simulink model "gm_uz_ninephase_VSD_transformation"  (R2021b)
settings: Solver=FixedStepAuto  StartTime=0.0  StopTime=inf  RelTol=1e-3
undefined symbols (not defined in the file or in its folder): a, b, c
libraries: hdlsllib x90, simulink x32, hdlmdlgenlib x20, dspsigops x7
(part 2 of 6)

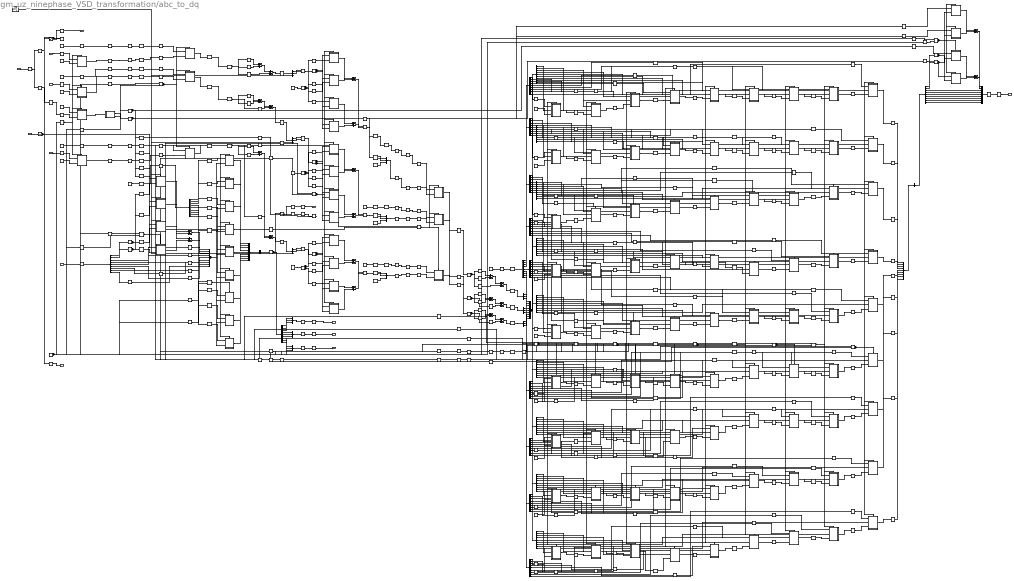
== system gm_uz_ninephase_VSD_transformation/abc_to_dq ==
  note: sin/cos calculation
  note: VSD and Park transformation
  note: VSD and Park inverse transformation
  note: Trigger Output
  x_in_dq : Inport  OutDataTypeStr=fixdt(1, 27, 18)  PortDimensions=[9]  SampleTime=1e-08
  theta_el : Inport  Port=2  OutDataTypeStr=fixdt(1, 18, 14)  PortDimensions=1  SampleTime=1e-08
  trigger_new_values : Inport  Port=3  OutDataTypeStr=boolean  PortDimensions=1  SampleTime=1e-08
  x_abc1_ll_pl : Inport  Port=4  OutDataTypeStr=fixdt(1, 27, 16)  PortDimensions=[3]  SampleTime=1e-08
  x_abc2_ll_pl : Inport  Port=5  OutDataTypeStr=fixdt(1, 27, 16)  PortDimensions=[3]  SampleTime=1e-08
  x_abc3_ll_pl : Inport  Port=6  OutDataTypeStr=fixdt(1, 27, 16)  PortDimensions=[3]  SampleTime=1e-08
  Add : Sum  AccumDataTypeStr=fixdt(1, 28, 16)  OutDataTypeStr=fixdt(1, 27, 16)  SampleTime=1e-10
  Add1 : Sum  AccumDataTypeStr=fixdt(1, 28, 18)  OutDataTypeStr=fixdt(1, 27, 18)  SampleTime=1e-10
  Add11 : Sum  Inputs=+-  AccumDataTypeStr=fixdt(1, 28, 16)  OutDataTypeStr=fixdt(1, 27, 16)  SampleTime=1e-10
  Add2 : Sum  Inputs=+-  AccumDataTypeStr=fixdt(1, 28, 18)  OutDataTypeStr=fixdt(1, 27, 18)  SampleTime=1e-10
  Complex to Real-Imag : ComplexToRealImag  SampleTime=1e-10
  Complex to Real-Imag1 : ComplexToRealImag  SampleTime=1e-10
  Complex to Real-Imag2 : ComplexToRealImag  SampleTime=1e-10
  Constant : Constant  Value=0  OutDataTypeStr=fixdt(1, 27, 16)  SampleTime=1e-10
  Constant1 : Constant  Value=[1;-0.5;-0.5;0.939697265625;-0.7660369873046875;-0.17364501953125;0.7660369873046875;-0.939697265625;0.17364501953125;0;0.86602783203125;-0.86602783203125;0.3420257568359375;0.642791748046875;-0.98480224609375;0.642791748046875;0.3420257568359375;-0.98480224609375;1;1;1;0.5;0.5;0.5;-0.5;-0.5;-0.5;0;0;0;0.86602783203125;0.86602783203125;0.86602783203125;0.86602783203125;0.86602783203125;0.86602783203125;1;-0.5;-0.5;-0.17364501953125;0.939697265625;-0.7660369873046875;-0.939697265625;0.17364501953125;0.7660369873046875;0;-0.86602783203125;0.86602783203125;0.98480224609375;-0.3420257568359375;-0.642791748046875;-0.3420257568359375;0.98480224609375;-0.642791748046875;1;-0.5;-0.5;-0.7660369873046875;-0.17364501953125;0.939697265625;0.17364501953125;0.7660369873046875;-0.939697265625;0;0.86602783203125;-0.86602783203125;0.642791748046875;-0.98480224609375;0.3420257568359375;-0.98480224609375;0.642791748046875;0.3420257568359375;1;1;1;-1;-1;-1;1;1;1]  OutDataTypeStr=fixdt(1, 18, 16)  SampleTime=1e-10
  Constant11 : Constant  Value=[0.22222137451171875;0;0.22222137451171875;0;0.22222137451171875;0;0.22222137451171875;0;0.111114501953125;-0.111114501953125;0.19245147705078125;0.22222137451171875;0;-0.111114501953125;-0.19245147705078125;-0.111114501953125;0.19245147705078125;0.111114501953125;-0.111114501953125;-0.19245147705078125;0.22222137451171875;0;-0.111114501953125;0.19245147705078125;-0.111114501953125;-0.19245147705078125;0.111114501953125;0.20882415771484375;0.0760040283203125;0.111114501953125;0.19245147705078125;-0.0385894775390625;0.21884918212890625;-0.17023468017578125;0.14284515380859375;-0.111114501953125;-0.17023468017578125;0.14284515380859375;0.111114501953125;0.19245147705078125;0.20882415771484375;-0.0760040283203125;-0.0385894775390625;-0.21884918212890625;-0.111114501953125;-0.0385894775390625;-0.21884918212890625;0.111114501953125;0.19245147705078125;-0.17023468017578125;-0.14284515380859375;0.20882415771484375;0.0760040283203125;-0.111114501953125;0.17023468017578125;0.14284515380859375;-0.111114501953125;0.19245147705078125;-0.20882415771484375;-0.0760040283203125;0.0385894775390625;-0.21884918212890625;0.111114501953125;-0.20882415771484375;0.0760040283203125;-0.111114501953125;0.19245147705078125;0.0385894775390625;0.21884918212890625;0.17023468017578125;0.14284515380859375;0.111114501953125;0.0385894775390625;-0.21884918212890625;-0.111114501953125;0.19245147705078125;0.17023468017578125;-0.14284515380859375;-0.20882415771484375;0.0760040283203125;0.111114501953125]  OutDataTypeStr=fixdt(1, 18, 17)  SampleTime=1e-10
  Constant12 : Constant  Value="fi(0,1,18,16,\"hex\",\"08000 + 3b619 i\")"  OutDataTypeStr=fixdt(1, 18, 16)  SampleTime=1e-10
  Constant13 : Constant  Value="fi(0,1,18,16,\"hex\",\"08000 + 3b619 i\")"  OutDataTypeStr=fixdt(1, 18, 16)  SampleTime=1e-10
  Constant14 : Constant  Value="fi(0,1,18,16,\"hex\",\"08000 + 3b619 i\")"  OutDataTypeStr=fixdt(1, 18, 16)  SampleTime=1e-10
  Constant2 : Constant  Value=0  OutDataTypeStr=fixdt(1, 27, 16)  SampleTime=1e-10
  Constant3 : Constant  Value=0  OutDataTypeStr=fixdt(1, 27, 16)  SampleTime=1e-10
  Delay9 : RateTransition  OutPortSampleTimeOpt=Multiple of input port sample time  OutPortSampleTimeMultiple=100
  Demux1_mux_1 : Mux  Inputs=3
  Demux1_mux_2 : Mux  Inputs=3
  Demux1_mux_3 : Mux  Inputs=3
  Demux1_out1 : Delay  DelayLength=double(1)  InitialCondition=0  SampleTime=1e-10
  Demux1_out2 : Delay  DelayLength=double(1)  InitialCondition=0  SampleTime=1e-10
  Demux1_out3 : Delay  DelayLength=double(1)  InitialCondition=0  SampleTime=1e-10
  Divide : Subsystem
      settings: MinAlgLoopOccurrences=on
  Divide1 : Subsystem
      settings: MinAlgLoopOccurrences=on
  Divide11 : Subsystem
      settings: MinAlgLoopOccurrences=on
  Divide2 : Subsystem
      settings: MinAlgLoopOccurrences=on
  Divide21 : Subsystem
      settings: MinAlgLoopOccurrences=on
  Divide3 : Subsystem
      settings: MinAlgLoopOccurrences=on
  Divide31 : Subsystem
      settings: MinAlgLoopOccurrences=on
  Divide4 : Subsystem
      settings: MinAlgLoopOccurrences=on
  From{,1..3,11..12,17..18,21..22} (10 alike) : hdlmdlgenlib/Buffer
      settings: SourceProductBaseCode=SL
  Gain : Subsystem
      settings: MinAlgLoopOccurrences=on
  Gain2 : Subsystem
      settings: MinAlgLoopOccurrences=on
  Gain21 : Subsystem
      settings: MinAlgLoopOccurrences=on
  Gain22 : Subsystem
      settings: MinAlgLoopOccurrences=on
  Gain2_const : Constant  Value=0.6666717529296875  OutDataTypeStr=fixdt(1, 18, 16)  SampleTime=1e-10
  Gain2_const1 : Constant  Value=0.6666717529296875  OutDataTypeStr=fixdt(1, 18, 16)  SampleTime=1e-10
  Gain2_const2 : Constant  Value=0.6666717529296875  OutDataTypeStr=fixdt(1, 18, 16)  SampleTime=1e-10
  Gain2_out_dtc : DataTypeConversion  OutDataTypeStr=fixdt(1, 27, 16)  SampleTime=1e-10  SaturateOnIntegerOverflow=on
  Gain2_out_dtc1 : DataTypeConversion  OutDataTypeStr=fixdt(1, 27, 16)  SampleTime=1e-10  SaturateOnIntegerOverflow=on
  Gain2_out_dtc2 : DataTypeConversion  OutDataTypeStr=fixdt(1, 27, 16)  SampleTime=1e-10  SaturateOnIntegerOverflow=on
  Gain4_const : Constant  Value=[1;0;0.5;-0.5;0.86602783203125;0.5;-0.5;-0.86602783203125;0.5]  OutDataTypeStr=fixdt(1, 18, 16)  SampleTime=1e-10
  Gain4_const1 : Constant  Value=[1;-0.5;-0.5;0;0.86602783203125;-0.86602783203125;1;1;1]  OutDataTypeStr=fixdt(1, 18, 16)  SampleTime=1e-10
  Gain4_const2 : Constant  Value=[1;0;0.5;-0.5;0.86602783203125;0.5;-0.5;-0.86602783203125;0.5]  OutDataTypeStr=fixdt(1, 18, 16)  SampleTime=1e-10
  Gain4_const3 : Constant  Value=[1;-0.5;-0.5;0;0.86602783203125;-0.86602783203125;1;1;1]  OutDataTypeStr=fixdt(1, 18, 16)  SampleTime=1e-10
  Gain4_const4 : Constant  Value=[1;0;0.5;-0.5;0.86602783203125;0.5;-0.5;-0.86602783203125;0.5]  OutDataTypeStr=fixdt(1, 18, 16)  SampleTime=1e-10
  Gain4_const5 : Constant  Value=[1;-0.5;-0.5;0;0.86602783203125;-0.86602783203125;1;1;1]  OutDataTypeStr=fixdt(1, 18, 16)  SampleTime=1e-10
  Gain_const : Constant  Value=0.1591548919677734375  OutDataTypeStr=fixdt(1, 18, 19)  SampleTime=1e-10
  Goto : hdlmdlgenlib/Buffer
      settings: SourceProductBaseCode=SL
  Goto1 : hdlmdlgenlib/Buffer
      settings: SourceProductBaseCode=SL
  Goto2 : hdlmdlgenlib/Buffer
      settings: SourceProductBaseCode=SL
  MMul_add_01 : Sum  OutDataTypeStr=fixdt(1, 27, 16)  SaturateOnIntegerOverflow=on  SampleTime=1e-10
  MMul_add_011 : Sum  OutDataTypeStr=fixdt(1, 27, 16)  SaturateOnIntegerOverflow=on  SampleTime=1e-10
  MMul_add_012 : Sum  OutDataTypeStr=fixdt(1, 27, 16)  SaturateOnIntegerOverflow=on  SampleTime=1e-10
  MMul_add_013 : Sum  OutDataTypeStr=fixdt(1, 27, 16)  SaturateOnIntegerOverflow=on  SampleTime=1e-10
  MMul_add_014 : Sum  OutDataTypeStr=fixdt(1, 27, 16)  SaturateOnIntegerOverflow=on  SampleTime=1e-10
  MMul_add_015 : Sum  OutDataTypeStr=fixdt(1, 27, 16)  SaturateOnIntegerOverflow=on  SampleTime=1e-10
  MMul_add_{12,121..125} (6 alike) : Sum  OutDataTypeStr=fixdt(1, 27, 16)  SaturateOnIntegerOverflow=on  SampleTime=1e-10
  MMul_dot_product : Subsystem
      settings: MinAlgLoopOccurrences=on
  MMul_dot_product1 : Subsystem
      settings: MinAlgLoopOccurrences=on
  MMul_dot_product2 : Subsystem
      settings: MinAlgLoopOccurrences=on
  MMul_dot_product3 : Subsystem
      settings: MinAlgLoopOccurrences=on
  MMul_dot_product4 : Subsystem
      settings: MinAlgLoopOccurrences=on
  MMul_dot_product5 : Subsystem
      settings: MinAlgLoopOccurrences=on
  MMul_dot_product_out_dtc{,1..5} (6 alike) : DataTypeConversion  OutDataTypeStr=fixdt(1, 27, 16)  SampleTime=1e-10  SaturateOnIntegerOverflow=on
  MatrixMultiply_out1_0_wire : hdlmdlgenlib/Buffer
      settings: SourceProductBaseCode=SL
  MatrixMultiply_out1_1_wire : hdlmdlgenlib/Buffer
      settings: SourceProductBaseCode=SL
  Product : Subsystem
      settings: MinAlgLoopOccurrences=on
  Product1 : Subsystem
      settings: MinAlgLoopOccurrences=on
  Product10 : Subsystem
      settings: MinAlgLoopOccurrences=on
  Product11 : Subsystem
      settings: MinAlgLoopOccurrences=on
  Product2 : Subsystem
      settings: MinAlgLoopOccurrences=on
  Product3 : Subsystem
      settings: MinAlgLoopOccurrences=on
  Product4 : Subsystem
      settings: MinAlgLoopOccurrences=on
  Product5 : Subsystem
      settings: MinAlgLoopOccurrences=on
  Product6 : Subsystem
      settings: MinAlgLoopOccurrences=on
  Product7 : Subsystem
      settings: MinAlgLoopOccurrences=on
  Product8 : Subsystem
      settings: MinAlgLoopOccurrences=on
  Product9 : Subsystem
      settings: MinAlgLoopOccurrences=on
  Product_AC_minus_BD : Sum  Inputs=+-  OutDataTypeStr=fixdt(1, 27, 16)  SampleTime=1e-10
  Product_AC_minus_BD1 : Sum  Inputs=+-  OutDataTypeStr=fixdt(1, 27, 16)  SampleTime=1e-10
  Product_AC_minus_BD2 : Sum  Inputs=+-  OutDataTypeStr=fixdt(1, 27, 16)  SampleTime=1e-10
  Product_AD_plus_BC : Sum  OutDataTypeStr=fixdt(1, 27, 16)  SampleTime=1e-10
  Product_AD_plus_BC1 : Sum  OutDataTypeStr=fixdt(1, 27, 16)  SampleTime=1e-10
  Product_AD_plus_BC2 : Sum  OutDataTypeStr=fixdt(1, 27, 16)  SampleTime=1e-10
  Product_C2ReIm_{1..2,11..12,21..22} (6 alike) : ComplexToRealImag  SampleTime=1e-10
  Product_ReIm2Complex : RealImagToComplex  SampleTime=1e-10
  Product_ReIm2Complex1 : RealImagToComplex  SampleTime=1e-10
  Product_ReIm2Complex2 : RealImagToComplex  SampleTime=1e-10
  Real-Imag to Complex : RealImagToComplex  ConstantPart="fi(0,1,27,16,\"hex\",\"0000000\")"  SampleTime=1e-10
  Real-Imag to Complex1 : RealImagToComplex  ConstantPart="fi(0,1,27,16,\"hex\",\"0000000\")"  SampleTime=1e-10
  Real-Imag to Complex2 : RealImagToComplex  ConstantPart="fi(0,1,27,16,\"hex\",\"0000000\")"  SampleTime=1e-10
  Reshape{,1..5} (6 alike) : Reshape  OutputDimensionality=Column vector (2-D)
  Row2Col_in{0..1,11..15} (7 alike) : Reshape  OutputDimensionality=Column vector (2-D)
  Row2Col_in01 : Reshape  OutputDimensionality=Column vector (2-D)
  Row2Col_in02 : Reshape  OutputDimensionality=Column vector (2-D)
  Row2Col_in03 : Reshape  OutputDimensionality=Column vector (2-D)
  Row2Col_in04 : Reshape  OutputDimensionality=Column vector (2-D)
  Row2Col_in05 : Reshape  OutputDimensionality=Column vector (2-D)
  Sine HDL Optimized : Subsystem  mask(Sine and Cosine HDL optimized block){OutputFormula=sin(2*pi*u) and cos(2*pi*u), NumDataPoints=double(256), TableDataTypeStr=fixdt(0,17,16), SimulateLUTROMDelay=off}
      mask prompts: OutputFormula "Simulink:masks:OutputFormula_MP"; NumDataPoints "HDLShared:hdlshared:CosineHDL_Npts"; TableDataTypeStr "Simulink:blkprm_prompts:TABLE_UNIFIEDDATATYPE"; SimulateLUTROMDelay "HDLShared:hdlshared:CosineHDL_SimulateLUTDelay"
      mask help: Sine and Cosine HDL optimized block using quarter wave symmetry, and HDL friendly settings.
      mask Help: helpview([docroot '/hdlcoder/helptargets.map'],'SineAndCosineHDL_Optimized');
      mask TypeOptions OutputFormula: sin(2*pi*u) | cos(2*pi*u) | exp(j*2*pi*u) | sin(2*pi*u) and cos(2*pi*u)
      mask Display:
      | port_label('input',1,'u')
      | port_label('output',1,'sin(2*pi*u)')
      | port_label('output',2,'cos(2*pi*u)')
      | xpos = 0.35;
      | yoffset = 0.5;
      | if ( SimulateLUTROMDelay )
      |   text(xpos,yoffset,'HDL (Z^{-1})','texmode','on')
      | else
      |    text(xpos,yoffset,'HDL')
      | end
  Switch : Switch  Criteria=u2 ~= 0  Threshold=double(0)  OutDataTypeStr=fixdt(1, 27, 18)  SampleTime=1e-10
  Switch1 : Switch  Criteria=u2 ~= 0  Threshold=double(0)  OutDataTypeStr=fixdt(1, 18, 14)  SampleTime=1e-08
  Switch_out1 : Delay  DelayLength=double(1)  InitialCondition=0  SampleTime=1e-10
  Switch_out11 : Delay  DelayLength=double(1)  InitialCondition=0  SampleTime=1e-10
  Transformation_out1 : Delay  DelayLength=double(1)  InitialCondition=0  SampleTime=1e-10
  Unit Delay : UnitDelay  SampleTime=1e-08
  _adder_MultiplyAdd : Subsystem
      settings: MinAlgLoopOccurrences=on
  _adder_MultiplyAdd1 : Subsystem
      settings: MinAlgLoopOccurrences=on
  _adder_MultiplyAdd10 : Subsystem
      settings: MinAlgLoopOccurrences=on
  _adder_MultiplyAdd11 : Subsystem
      settings: MinAlgLoopOccurrences=on
  _adder_MultiplyAdd12 : Subsystem
      settings: MinAlgLoopOccurrences=on
  _adder_MultiplyAdd13 : Subsystem
      settings: MinAlgLoopOccurrences=on
  _adder_MultiplyAdd14 : Subsystem
      settings: MinAlgLoopOccurrences=on
  _adder_MultiplyAdd15 : Subsystem
      settings: MinAlgLoopOccurrences=on
  _adder_MultiplyAdd16 : Subsystem
      settings: MinAlgLoopOccurrences=on
  _adder_MultiplyAdd17 : Subsystem
      settings: MinAlgLoopOccurrences=on
  _adder_MultiplyAdd18 : Subsystem
      settings: MinAlgLoopOccurrences=on
  _adder_MultiplyAdd19 : Subsystem
      settings: MinAlgLoopOccurrences=on
  _adder_MultiplyAdd2 : Subsystem
      settings: MinAlgLoopOccurrences=on
  _adder_MultiplyAdd20 : Subsystem
      settings: MinAlgLoopOccurrences=on
  _adder_MultiplyAdd21 : Subsystem
      settings: MinAlgLoopOccurrences=on
  _adder_MultiplyAdd22 : Subsystem
      settings: MinAlgLoopOccurrences=on
  _adder_MultiplyAdd23 : Subsystem
      settings: MinAlgLoopOccurrences=on
  _adder_MultiplyAdd24 : Subsystem
      settings: MinAlgLoopOccurrences=on
  _adder_MultiplyAdd25 : Subsystem
      settings: MinAlgLoopOccurrences=on
  _adder_MultiplyAdd26 : Subsystem
      settings: MinAlgLoopOccurrences=on
  _adder_MultiplyAdd27 : Subsystem
      settings: MinAlgLoopOccurrences=on
  _adder_MultiplyAdd28 : Subsystem
      settings: MinAlgLoopOccurrences=on
  _adder_MultiplyAdd29 : Subsystem
      settings: MinAlgLoopOccurrences=on
  _adder_MultiplyAdd3 : Subsystem
      settings: MinAlgLoopOccurrences=on
  _adder_MultiplyAdd30 : Subsystem
      settings: MinAlgLoopOccurrences=on
  _adder_MultiplyAdd31 : Subsystem
      settings: MinAlgLoopOccurrences=on
  _adder_MultiplyAdd32 : Subsystem
      settings: MinAlgLoopOccurrences=on
  _adder_MultiplyAdd33 : Subsystem
      settings: MinAlgLoopOccurrences=on
  _adder_MultiplyAdd34 : Subsystem
      settings: MinAlgLoopOccurrences=on
  _adder_MultiplyAdd35 : Subsystem
      settings: MinAlgLoopOccurrences=on
  _adder_MultiplyAdd36 : Subsystem
      settings: MinAlgLoopOccurrences=on
  _adder_MultiplyAdd37 : Subsystem
      settings: MinAlgLoopOccurrences=on
  _adder_MultiplyAdd38 : Subsystem
      settings: MinAlgLoopOccurrences=on
  _adder_MultiplyAdd39 : Subsystem
      settings: MinAlgLoopOccurrences=on
  _adder_MultiplyAdd4 : Subsystem
      settings: MinAlgLoopOccurrences=on
  _adder_MultiplyAdd40 : Subsystem
      settings: MinAlgLoopOccurrences=on
  _adder_MultiplyAdd41 : Subsystem
      settings: MinAlgLoopOccurrences=on
  _adder_MultiplyAdd42 : Subsystem
      settings: MinAlgLoopOccurrences=on
  _adder_MultiplyAdd43 : Subsystem
      settings: MinAlgLoopOccurrences=on
  _adder_MultiplyAdd44 : Subsystem
      settings: MinAlgLoopOccurrences=on
  _adder_MultiplyAdd45 : Subsystem
      settings: MinAlgLoopOccurrences=on
  _adder_MultiplyAdd46 : Subsystem
      settings: MinAlgLoopOccurrences=on
  _adder_MultiplyAdd47 : Subsystem
      settings: MinAlgLoopOccurrences=on
  _adder_MultiplyAdd48 : Subsystem
      settings: MinAlgLoopOccurrences=on
  _adder_MultiplyAdd49 : Subsystem
      settings: MinAlgLoopOccurrences=on
  _adder_MultiplyAdd5 : Subsystem
      settings: MinAlgLoopOccurrences=on
  _adder_MultiplyAdd50 : Subsystem
      settings: MinAlgLoopOccurrences=on
  _adder_MultiplyAdd51 : Subsystem
      settings: MinAlgLoopOccurrences=on
  _adder_MultiplyAdd52 : Subsystem
      settings: MinAlgLoopOccurrences=on
  _adder_MultiplyAdd53 : Subsystem
      settings: MinAlgLoopOccurrences=on
  _adder_MultiplyAdd54 : Subsystem
      settings: MinAlgLoopOccurrences=on
  _adder_MultiplyAdd55 : Subsystem
      settings: MinAlgLoopOccurrences=on
  _adder_MultiplyAdd56 : Subsystem
      settings: MinAlgLoopOccurrences=on
  _adder_MultiplyAdd57 : Subsystem
      settings: MinAlgLoopOccurrences=on
  _adder_MultiplyAdd58 : Subsystem
      settings: MinAlgLoopOccurrences=on
  _adder_MultiplyAdd59 : Subsystem
      settings: MinAlgLoopOccurrences=on
  _adder_MultiplyAdd6 : Subsystem
      settings: MinAlgLoopOccurrences=on
  _adder_MultiplyAdd60 : Subsystem
      settings: MinAlgLoopOccurrences=on
  _adder_MultiplyAdd61 : Subsystem
      settings: MinAlgLoopOccurrences=on
  _adder_MultiplyAdd62 : Subsystem
      settings: MinAlgLoopOccurrences=on
  _adder_MultiplyAdd63 : Subsystem
      settings: MinAlgLoopOccurrences=on
  _adder_MultiplyAdd64 : Subsystem
      settings: MinAlgLoopOccurrences=on
  _adder_MultiplyAdd65 : Subsystem
      settings: MinAlgLoopOccurrences=on
  _adder_MultiplyAdd66 : Subsystem
      settings: MinAlgLoopOccurrences=on
  _adder_MultiplyAdd67 : Subsystem
      settings: MinAlgLoopOccurrences=on
  _adder_MultiplyAdd68 : Subsystem
      settings: MinAlgLoopOccurrences=on
  _adder_MultiplyAdd69 : Subsystem
      settings: MinAlgLoopOccurrences=on
  _adder_MultiplyAdd7 : Subsystem
      settings: MinAlgLoopOccurrences=on
  _adder_MultiplyAdd70 : Subsystem
      settings: MinAlgLoopOccurrences=on
  _adder_MultiplyAdd71 : Subsystem
      settings: MinAlgLoopOccurrences=on
  _adder_MultiplyAdd72 : Subsystem
      settings: MinAlgLoopOccurrences=on
  _adder_MultiplyAdd73 : Subsystem
      settings: MinAlgLoopOccurrences=on
  _adder_MultiplyAdd74 : Subsystem
      settings: MinAlgLoopOccurrences=on
  _adder_MultiplyAdd75 : Subsystem
      settings: MinAlgLoopOccurrences=on
  _adder_MultiplyAdd76 : Subsystem
      settings: MinAlgLoopOccurrences=on
  _adder_MultiplyAdd77 : Subsystem
      settings: MinAlgLoopOccurrences=on
  _adder_MultiplyAdd78 : Subsystem
      settings: MinAlgLoopOccurrences=on
  _adder_MultiplyAdd79 : Subsystem
      settings: MinAlgLoopOccurrences=on
  _adder_MultiplyAdd8 : Subsystem
      settings: MinAlgLoopOccurrences=on
  _adder_MultiplyAdd80 : Subsystem
      settings: MinAlgLoopOccurrences=on
  _adder_MultiplyAdd9 : Subsystem
      settings: MinAlgLoopOccurrences=on
  _adder_MultiplyAdd_out_dtc{,1..80} (81 alike) : DataTypeConversion  OutDataTypeStr=fixdt(1, 27, 16)  SampleTime=1e-10
  _bias{,1..8} (9 alike) : Constant  Value=double(0)  OutDataTypeStr=fixdt(1, 27, 16)  SampleTime=1e-10
  abc   to   alpha_beta_0_out1_2_term2 : Terminator
  abc   to   alpha_beta_0_out1_2_term21 : Terminator
  abc   to   alpha_beta_0_out1_2_term22 : Terminator
  crp_temp_MAC : Subsystem
      settings: MinAlgLoopOccurrences=on
  crp_temp_MAC1 : Subsystem
      settings: MinAlgLoopOccurrences=on
  crp_temp_MAC2 : Subsystem
      settings: MinAlgLoopOccurrences=on
  crp_temp_MAC3 : Subsystem
      settings: MinAlgLoopOccurrences=on
  crp_temp_MAC4 : Subsystem
      settings: MinAlgLoopOccurrences=on
  crp_temp_MAC5 : Subsystem
      settings: MinAlgLoopOccurrences=on
  crp_temp_MAC6 : Subsystem
      settings: MinAlgLoopOccurrences=on
  crp_temp_MAC7 : Subsystem
      settings: MinAlgLoopOccurrences=on
  crp_temp_MAC8 : Subsystem
      settings: MinAlgLoopOccurrences=on
  ctr_99 : simulink/Sources/Counter Limited  uplimit=double(99)  tsamp=1e-10
  delayMatch{,1,121..122} (4 alike) : Delay  DelayLength=double(1)  InitialCondition=0  SampleTime=1e-08
  delayMatch{2..21,23..27,29..33,35..120} (116 alike) : Delay  DelayLength=double(1)  InitialCondition=0  SampleTime=1e-10
  delayMatch22 : Delay  DelayLength=double(2)  InitialCondition=0  SampleTime=1e-10
  delayMatch28 : Delay  DelayLength=double(2)  InitialCondition=0  SampleTime=1e-10
  delayMatch34 : Delay  DelayLength=double(2)  InitialCondition=0  SampleTime=1e-10
  enb_counter_ge_11 : simulink/Logic and Bit Operations/Compare To Constant  relop=>=  const=double(11)  OutDataTypeStr=boolean
  enb_counter_ge_11_and_enb_counter_le_14 : Logic  AllPortsSameDT=off  OutDataTypeStr=boolean  SampleTime=1e-10
  enb_counter_ge_14 : simulink/Logic and Bit Operations/Compare To Constant  relop=>=  const=double(14)  OutDataTypeStr=boolean
  enb_counter_ge_14_and_enb_counter_le_17 : Logic  AllPortsSameDT=off  OutDataTypeStr=boolean  SampleTime=1e-10
  enb_counter_ge_17 : simulink/Logic and Bit Operations/Compare To Constant  relop=>=  const=double(17)  OutDataTypeStr=boolean
  enb_counter_ge_17_and_enb_counter_le_20 : Logic  AllPortsSameDT=off  OutDataTypeStr=boolean  SampleTime=1e-10
  enb_counter_ge_2 : simulink/Logic and Bit Operations/Compare To Constant  relop=>=  const=double(2)  OutDataTypeStr=boolean
  enb_counter_ge_20 : simulink/Logic and Bit Operations/Compare To Constant  relop=>=  const=double(20)  OutDataTypeStr=boolean
  enb_counter_ge_20_and_enb_counter_le_23 : Logic  AllPortsSameDT=off  OutDataTypeStr=boolean  SampleTime=1e-10
  enb_counter_ge_23 : simulink/Logic and Bit Operations/Compare To Constant  relop=>=  const=double(23)  OutDataTypeStr=boolean
  enb_counter_ge_23_and_enb_counter_le_26 : Logic  AllPortsSameDT=off  OutDataTypeStr=boolean  SampleTime=1e-10
  enb_counter_ge_26 : simulink/Logic and Bit Operations/Compare To Constant  relop=>=  const=double(26)  OutDataTypeStr=boolean
  enb_counter_ge_26_and_enb_counter_le_29 : Logic  AllPortsSameDT=off  OutDataTypeStr=boolean  SampleTime=1e-10
  enb_counter_ge_29 : simulink/Logic and Bit Operations/Compare To Constant  relop=>=  const=double(29)  OutDataTypeStr=boolean
  enb_counter_ge_29_and_enb_counter_le_32 : Logic  AllPortsSameDT=off  OutDataTypeStr=boolean  SampleTime=1e-10
  enb_counter_ge_2_and_enb_counter_le_4 : Logic  AllPortsSameDT=off  OutDataTypeStr=boolean  SampleTime=1e-10
  enb_counter_ge_3 : simulink/Logic and Bit Operations/Compare To Constant  relop=>=  const=double(3)  OutDataTypeStr=boolean
  enb_counter_ge_32 : simulink/Logic and Bit Operations/Compare To Constant  relop=>=  const=double(32)  OutDataTypeStr=boolean
  enb_counter_ge_32_and_enb_counter_le_35 : Logic  AllPortsSameDT=off  OutDataTypeStr=boolean  SampleTime=1e-10
  enb_counter_ge_35 : simulink/Logic and Bit Operations/Compare To Constant  relop=>=  const=double(35)  OutDataTypeStr=boolean
  enb_counter_ge_35_and_enb_counter_le_37 : Logic  AllPortsSameDT=off  OutDataTypeStr=boolean  SampleTime=1e-10
  enb_counter_ge_3_and_enb_counter_le_5 : Logic  AllPortsSameDT=off  OutDataTypeStr=boolean  SampleTime=1e-10
  enb_counter_ge_4 : simulink/Logic and Bit Operations/Compare To Constant  relop=>=  const=double(4)  OutDataTypeStr=boolean
  enb_counter_ge_4_and_enb_counter_le_6 : Logic  AllPortsSameDT=off  OutDataTypeStr=boolean  SampleTime=1e-10
  enb_counter_ge_5 : simulink/Logic and Bit Operations/Compare To Constant  relop=>=  const=double(5)  OutDataTypeStr=boolean
  enb_counter_ge_5_and_enb_counter_le_13 : Logic  AllPortsSameDT=off  OutDataTypeStr=boolean  SampleTime=1e-10
  enb_counter_ge_6 : simulink/Logic and Bit Operations/Compare To Constant  relop=>=  const=double(6)  OutDataTypeStr=boolean
  enb_counter_ge_6_and_enb_counter_le_8 : Logic  AllPortsSameDT=off  OutDataTypeStr=boolean  SampleTime=1e-10
  enb_counter_ge_8 : simulink/Logic and Bit Operations/Compare To Constant  relop=>=  const=double(8)  OutDataTypeStr=boolean
  enb_counter_ge_8_and_enb_counter_le_11 : Logic  AllPortsSameDT=off  OutDataTypeStr=boolean  SampleTime=1e-10
  enb_counter_le_11 : simulink/Logic and Bit Operations/Compare To Constant  relop=<=  const=double(11)  OutDataTypeStr=boolean
  enb_counter_le_13 : simulink/Logic and Bit Operations/Compare To Constant  relop=<=  const=double(13)  OutDataTypeStr=boolean
  enb_counter_le_14 : simulink/Logic and Bit Operations/Compare To Constant  relop=<=  const=double(14)  OutDataTypeStr=boolean
  enb_counter_le_17 : simulink/Logic and Bit Operations/Compare To Constant  relop=<=  const=double(17)  OutDataTypeStr=boolean
  enb_counter_le_2 : simulink/Logic and Bit Operations/Compare To Constant  relop=<=  const=double(2)  OutDataTypeStr=boolean
  enb_counter_le_20 : simulink/Logic and Bit Operations/Compare To Constant  relop=<=  const=double(20)  OutDataTypeStr=boolean
  enb_counter_le_23 : simulink/Logic and Bit Operations/Compare To Constant  relop=<=  const=double(23)  OutDataTypeStr=boolean
  enb_counter_le_26 : simulink/Logic and Bit Operations/Compare To Constant  relop=<=  const=double(26)  OutDataTypeStr=boolean
  enb_counter_le_29 : simulink/Logic and Bit Operations/Compare To Constant  relop=<=  const=double(29)  OutDataTypeStr=boolean
  enb_counter_le_32 : simulink/Logic and Bit Operations/Compare To Constant  relop=<=  const=double(32)  OutDataTypeStr=boolean
  enb_counter_le_35 : simulink/Logic and Bit Operations/Compare To Constant  relop=<=  const=double(35)  OutDataTypeStr=boolean
  enb_counter_le_37 : simulink/Logic and Bit Operations/Compare To Constant  relop=<=  const=double(37)  OutDataTypeStr=boolean
  enb_counter_le_4 : simulink/Logic and Bit Operations/Compare To Constant  relop=<=  const=double(4)  OutDataTypeStr=boolean
  enb_counter_le_5 : simulink/Logic and Bit Operations/Compare To Constant  relop=<=  const=double(5)  OutDataTypeStr=boolean
  enb_counter_le_6 : simulink/Logic and Bit Operations/Compare To Constant  relop=<=  const=double(6)  OutDataTypeStr=boolean
  enb_counter_le_8 : simulink/Logic and Bit Operations/Compare To Constant  relop=<=  const=double(8)  OutDataTypeStr=boolean
  in0_repeat : dspsigops/Repeat  N=double(100)  RateOptions=Allow multirate processing  ic=0  mode=Unused parameter value
  in1_repeat : dspsigops/Repeat  N=double(100)  RateOptions=Allow multirate processing  ic=0  mode=Unused parameter value
  in2_repeat : dspsigops/Repeat  N=double(100)  RateOptions=Allow multirate processing  ic=0  mode=Unused parameter value
  in3_repeat : dspsigops/Repeat  N=double(100)  RateOptions=Allow multirate processing  ic=0  mode=Unused parameter value
  in4_repeat : dspsigops/Repeat  N=double(100)  RateOptions=Allow multirate processing  ic=0  mode=Unused parameter value
  in5_repeat : dspsigops/Repeat  N=double(100)  RateOptions=Allow multirate processing  ic=0  mode=Unused parameter value
  in6_repeat : dspsigops/Repeat  N=double(100)  RateOptions=Allow multirate processing  ic=0  mode=Unused parameter value
  inverse Transformation_out1 : hdlmdlgenlib/Buffer
      settings: SourceProductBaseCode=SL
  mux : Mux  Inputs=3
  mux1 : Mux  Inputs=3
  mux2 : Mux  Inputs=3
  mux3 : Mux  Inputs=9
  mux4 : Mux  Inputs=9
  mux5 : Mux  Inputs=9
  reshape_dotProduct{,1..5} (6 alike) : Reshape  OutputDimensionality=Customize  OutputDimensions=[3,3]
  reshape_mmulResult{,1..5} (6 alike) : Reshape  OutputDimensionality=Customize  OutputDimensions=[3,1]
  select_0 : Selector  NumberOfDimensions=2  SampleTime=1e-10  IndexOptions=Index vector (dialog),Select all  Indices=double(1),[]  OutputSizes=1
  select_01 : Selector  NumberOfDimensions=2  SampleTime=1e-10  IndexOptions=Index vector (dialog),Select all  Indices=double(1),[]  OutputSizes=1
  select_02 : Selector  NumberOfDimensions=2  SampleTime=1e-10  IndexOptions=Index vector (dialog),Select all  Indices=double(1),[]  OutputSizes=1
  select_03 : Selector  NumberOfDimensions=2  SampleTime=1e-10  IndexOptions=Index vector (dialog),Select all  Indices=double(1),[]  OutputSizes=1
  select_04 : Selector  NumberOfDimensions=2  SampleTime=1e-10  IndexOptions=Index vector (dialog),Select all  Indices=double(1),[]  OutputSizes=1
  select_05 : Selector  NumberOfDimensions=2  SampleTime=1e-10  IndexOptions=Index vector (dialog),Select all  Indices=double(1),[]  OutputSizes=1
  select_{1,11..15} (6 alike) : Selector  NumberOfDimensions=2  SampleTime=1e-10  IndexOptions=Index vector (dialog),Select all  Indices=double(2),[]  OutputSizes=1
  select_{2,21..25} (6 alike) : Selector  NumberOfDimensions=2  SampleTime=1e-10  IndexOptions=Index vector (dialog),Select all  Indices=double(3),[]  OutputSizes=1
  select_indices0 : Selector  SampleTime=1e-10  IndexOptions=Index vector (dialog)  Indices=double([1 4 7 2 5 8 3 6 9])  OutputSizes=1
  select_indices01 : Selector  SampleTime=1e-10  IndexOptions=Index vector (dialog)  Indices=double([1 4 7 2 5 8 3 6 9])  OutputSizes=1
  select_indices02 : Selector  SampleTime=1e-10  IndexOptions=Index vector (dialog)  Indices=double([1 4 7 2 5 8 3 6 9])  OutputSizes=1
  select_indices03 : Selector  SampleTime=1e-10  IndexOptions=Index vector (dialog)  Indices=double([1 4 7 2 5 8 3 6 9])  OutputSizes=1
  select_indices04 : Selector  SampleTime=1e-10  IndexOptions=Index vector (dialog)  Indices=double([1 4 7 2 5 8 3 6 9])  OutputSizes=1
  select_indices05 : Selector  SampleTime=1e-10  IndexOptions=Index vector (dialog)  Indices=double([1 4 7 2 5 8 3 6 9])  OutputSizes=1
  select_indices{1,11..15} (6 alike) : Selector  SampleTime=1e-10  IndexOptions=Index vector (dialog)  Indices=double([1 2 3 1 2 3 1 2 3])  OutputSizes=1
  t{,7..8,25..42} (21 alike) : Demux  Outputs=9
  t{1..6} (6 alike) : Demux  Outputs=3
  t10 : Reshape  OutputDimensionality=Customize  OutputDimensions=[9,9]
  t{11..16} (6 alike) : Reshape  OutputDimensionality=Customize  OutputDimensions=[3,3]
  t17 : Math  Operator=transpose  SaturateOnIntegerOverflow=on
  t18 : Subsystem
  t19 : Mux  Inputs=9
  t20 : Concatenate  NumInputs=1  Mode=Multidimensional array  ConcatenateDimension=2
  t21 : Math  Operator=transpose  SaturateOnIntegerOverflow=on
  t22 : Subsystem
  t23 : Mux  Inputs=9
  t24 : Concatenate  NumInputs=1  Mode=Multidimensional array  ConcatenateDimension=2
  t{43..47} (5 alike) : RateTransition  OutPortSampleTimeOpt=Multiple of input port sample time  OutPortSampleTimeMultiple=100
  t9 : Reshape  OutputDimensionality=Customize  OutputDimensions=[9,9]
  vectorized_in0 : Reshape  OutputDimensionality=Row vector (2-D)
  vectorized_in01 : Reshape  OutputDimensionality=Row vector (2-D)
  vectorized_in02 : Reshape  OutputDimensionality=Row vector (2-D)
  vectorized_in03 : Reshape  OutputDimensionality=Row vector (2-D)
  vectorized_in04 : Reshape  OutputDimensionality=Row vector (2-D)
  vectorized_in05 : Reshape  OutputDimensionality=Row vector (2-D)
  x_in_dq_0_wire : hdlmdlgenlib/Buffer
      settings: SourceProductBaseCode=SL
  x_in_dq_1_wire : hdlmdlgenlib/Buffer
      settings: SourceProductBaseCode=SL
  theta_el_axi : Outport  SampleTime=1e-08
  x_abc_out_axi : Outport  Port=2  SampleTime=1e-08
  x_abc_1 : Outport  Port=3  SampleTime=1e-08
  x_abc_2 : Outport  Port=4  SampleTime=1e-08
  x_abc_3 : Outport  Port=5  SampleTime=1e-08
  x_out_dq : Outport  Port=6  SampleTime=1e-08
  refresh_values : Outport  Port=7  SampleTime=1e-08
  wires:
  x_in_dq/1 -> in2_repeat/1
  theta_el/1 -> Goto2/1
  trigger_new_values/1 -> Unit Delay/1
  x_abc1_ll_pl/1 -> in4_repeat/1
  x_abc2_ll_pl/1 -> in5_repeat/1
  x_abc3_ll_pl/1 -> in6_repeat/1
  delayMatch1/1 -> in3_repeat/1
  delayMatch122/1 -> refresh_values/1
  delayMatch121/1 -> theta_el_axi/1
  t43/1 -> x_abc_1/1
  t44/1 -> x_abc_2/1
  t45/1 -> x_abc_3/1
  t46/1 -> x_abc_out_axi/1
  t47/1 -> x_out_dq/1
  Switch1/1 -> delayMatch121/1, delayMatch/1
  Unit Delay/1 -> delayMatch122/1, Switch1/2, in0_repeat/1
  delayMatch/1 -> Switch1/3
  Delay9/1 -> in1_repeat/1
  Goto2/1 -> From1/1, From/1
  From1/1 -> Switch1/1
  From/1 -> delayMatch1/1
  Demux1_out1/1 -> t43/1
  Demux1_out2/1 -> t44/1
  Demux1_out3/1 -> t45/1
  Switch_out1/1 -> Delay9/1
  Switch_out11/1 -> t46/1
  Transformation_out1/1 -> t47/1
  in0_repeat/1 -> Switch/2
  in1_repeat/1 -> Switch/3
  in2_repeat/1 -> t/1
  in3_repeat/1 -> Gain/2(in1)
  in4_repeat/1 -> Gain2/1(in0)
  in5_repeat/1 -> Gain21/1(in0)
  in6_repeat/1 -> Gain22/1(in0)
  t9/1 -> t21/1
  Divide1/1(out0) -> Add/2
  From21/1 -> Divide3/1(in0)
  Divide3/1(out0) -> Add1/2
  Add1/1 -> mux5/2
  From11/1 -> Divide2/1(in0)
  Divide2/1(out0) -> Add1/1
  delayMatch2/1 -> Divide4/2(in1)
  delayMatch4/1 -> Divide11/2(in1)
  delayMatch6/1 -> mux5/3
  delayMatch7/1 -> mux5/4
  delayMatch8/1 -> mux5/5
  delayMatch9/1 -> mux5/6
  delayMatch10/1 -> mux5/7
  delayMatch11/1 -> mux5/8
  delayMatch12/1 -> mux5/9
  Divide11/1(out0) -> Add2/2
  From18/1 -> Divide11/1(in0)
  Gain/1(out0) -> Sine HDL Optimized/1(u)
  Sine HDL Optimized/1(x) -> Goto/1
  Sine HDL Optimized/2(y) -> Goto1/1
  Goto/1 -> From3/1, From12/1, From18/1, From11/1
  Divide21/1(out0) -> Add11/2
  t10/1 -> t17/1
  Gain2_out_dtc/1 -> Reshape/1
  Reshape/1 -> select_indices1/1
  reshape_mmulResult/1 -> t1/1
  Real-Imag to Complex/1 -> Product_C2ReIm_1/1
  Constant12/1 -> Product_C2ReIm_2/1
  Product_ReIm2Complex/1 -> Complex to Real-Imag/1
  Complex to Real-Imag/1 -> mux/1
  Complex to Real-Imag/2 -> mux/2
  Constant/1 -> mux/3
  mux/1 -> Reshape1/1
  Reshape1/1 -> select_indices11/1
  reshape_mmulResult1/1 -> t4/1
  Gain2_out_dtc1/1 -> Reshape2/1
  Reshape2/1 -> select_indices12/1
  reshape_mmulResult2/1 -> t2/1
  Real-Imag to Complex1/1 -> Product_C2ReIm_11/1
  Constant13/1 -> Product_C2ReIm_21/1
  Product_ReIm2Complex1/1 -> Complex to Real-Imag1/1
  Complex to Real-Imag1/1 -> mux1/1
  Complex to Real-Imag1/2 -> mux1/2
  Constant2/1 -> mux1/3
  mux1/1 -> Reshape3/1
  Reshape3/1 -> select_indices13/1
  reshape_mmulResult3/1 -> t5/1
  Gain2_out_dtc2/1 -> Reshape4/1
  Reshape4/1 -> select_indices14/1
  reshape_mmulResult4/1 -> t3/1
  Real-Imag to Complex2/1 -> Product_C2ReIm_12/1
  Constant14/1 -> Product_C2ReIm_22/1
  Product_ReIm2Complex2/1 -> Complex to Real-Imag2/1
  Complex to Real-Imag2/1 -> mux2/1
  Complex to Real-Imag2/2 -> mux2/2
  Constant3/1 -> mux2/3
  mux2/1 -> Reshape5/1
  Reshape5/1 -> select_indices15/1
  reshape_mmulResult5/1 -> t6/1
  mux3/1 -> t42/1, t40/1, t38/1, t36/1, t34/1, t32/1, t30/1, t28/1, t26/1
  t20/1 -> t7/1
  MatrixMultiply_out1_0_wire/1 -> Divide/2(in1), Divide21/2(in1)
  MatrixMultiply_out1_1_wire/1 -> Divide1/2(in1), Divide31/2(in1)
  Divide/1(out0) -> Add/1
  Add/1 -> mux4/1
  mux4/1 -> Transformation_out1/1
  Add11/1 -> mux4/2
  Divide31/1(out0) -> Add11/1
  Goto1/1 -> From22/1, From2/1, From21/1, From17/1
  From17/1 -> Divide4/1(in0)
  Divide4/1(out0) -> Add2/1
  Add2/1 -> mux5/1
  mux5/1 -> crp_temp_MAC2/2(in1), crp_temp_MAC1/2(in1), crp_temp_MAC5/2(in1), crp_temp_MAC6/2(in1), crp_temp_MAC7/2(in1), crp_temp_MAC8/2(in1), crp_temp_MAC/2(in1), crp_temp_MAC3/2(in1), crp_temp_MAC4/2(in1)
  t24/1 -> inverse Transformation_out1/1
  inverse Transformation_out1/1 -> t8/1, Switch/1
  t/1 -> x_in_dq_0_wire/1
  t/2 -> x_in_dq_1_wire/1
  t/3 -> delayMatch6/1
  t/4 -> delayMatch7/1
  t/5 -> delayMatch8/1
  t/6 -> delayMatch9/1
  t/7 -> delayMatch10/1
  t/8 -> delayMatch11/1
  t/9 -> delayMatch12/1
  t1/1 -> Real-Imag to Complex/1
  t1/2 -> Real-Imag to Complex/2
  t1/3 -> abc   to   alpha_beta_0_out1_2_term21/1
  t2/1 -> Real-Imag to Complex1/1
  t2/2 -> Real-Imag to Complex1/2
  t2/3 -> abc   to   alpha_beta_0_out1_2_term22/1
  t3/1 -> Real-Imag to Complex2/1
  t3/2 -> Real-Imag to Complex2/2
  t3/3 -> abc   to   alpha_beta_0_out1_2_term2/1
  t4/1 -> mux3/1
  t4/2 -> mux3/2
  t4/3 -> mux3/3
  t5/1 -> mux3/4
  t5/2 -> mux3/5
  t5/3 -> mux3/6
  t6/1 -> mux3/7
  t6/2 -> mux3/8
  t6/3 -> mux3/9
  t7/1 -> MatrixMultiply_out1_0_wire/1
  t7/2 -> MatrixMultiply_out1_1_wire/1
  t7/3 -> mux4/3
  t7/4 -> mux4/4
  t7/5 -> mux4/5
  t7/6 -> mux4/6
  t7/7 -> mux4/7
  t7/8 -> mux4/8
  t7/9 -> mux4/9
  t8/1 -> Demux1_mux_1/1
  t8/2 -> Demux1_mux_1/2
  t8/3 -> Demux1_mux_1/3
  t8/4 -> Demux1_mux_2/1
  t8/5 -> Demux1_mux_2/2
  t8/6 -> Demux1_mux_2/3
  t8/7 -> Demux1_mux_3/1
  t8/8 -> Demux1_mux_3/2
  t8/9 -> Demux1_mux_3/3
  Constant1/1 -> t9/1
  Constant11/1 -> t10/1
  t11/1 -> vectorized_in0/1
  vectorized_in0/1 -> select_indices0/1
  select_indices0/1 -> Row2Col_in0/1
  select_indices1/1 -> Row2Col_in1/1
  delayMatch22/1 -> MMul_dot_product/1(in0)
  Row2Col_in1/1 -> MMul_dot_product/2(in1)
  MMul_dot_product_out_dtc/1 -> reshape_dotProduct/1
  reshape_dotProduct/1 -> select_2/1, select_1/1, select_0/1
  select_0/1 -> MMul_add_01/1
  select_1/1 -> MMul_add_01/2
  MMul_add_01/1 -> MMul_add_12/1
  select_2/1 -> MMul_add_12/2
  MMul_add_12/1 -> reshape_mmulResult/1
  Gain4_const/1 -> t11/1
  t12/1 -> vectorized_in01/1
  vectorized_in01/1 -> select_indices01/1
  select_indices01/1 -> Row2Col_in01/1
  select_indices11/1 -> Row2Col_in11/1
  delayMatch27/1 -> MMul_dot_product1/1(in0)
  Row2Col_in11/1 -> MMul_dot_product1/2(in1)
  MMul_dot_product_out_dtc1/1 -> reshape_dotProduct1/1
  reshape_dotProduct1/1 -> select_21/1, select_11/1, select_01/1
  select_01/1 -> MMul_add_011/1
  select_11/1 -> MMul_add_011/2
  MMul_add_011/1 -> MMul_add_121/1
  select_21/1 -> MMul_add_121/2
  MMul_add_121/1 -> reshape_mmulResult1/1
  Gain4_const1/1 -> t12/1
  t13/1 -> vectorized_in02/1
  vectorized_in02/1 -> select_indices02/1
  select_indices02/1 -> Row2Col_in02/1
  select_indices12/1 -> Row2Col_in12/1
  delayMatch28/1 -> MMul_dot_product2/1(in0)
  Row2Col_in12/1 -> MMul_dot_product2/2(in1)
  MMul_dot_product_out_dtc2/1 -> reshape_dotProduct2/1
  reshape_dotProduct2/1 -> select_22/1, select_12/1, select_02/1
  select_02/1 -> MMul_add_012/1
  select_12/1 -> MMul_add_012/2
  MMul_add_012/1 -> MMul_add_122/1
  select_22/1 -> MMul_add_122/2
  MMul_add_122/1 -> reshape_mmulResult2/1
  Gain4_const2/1 -> t13/1
  t14/1 -> vectorized_in03/1
  vectorized_in03/1 -> select_indices03/1
  select_indices03/1 -> Row2Col_in03/1
  select_indices13/1 -> Row2Col_in13/1
  delayMatch33/1 -> MMul_dot_product3/1(in0)
  Row2Col_in13/1 -> MMul_dot_product3/2(in1)
  MMul_dot_product_out_dtc3/1 -> reshape_dotProduct3/1
  reshape_dotProduct3/1 -> select_23/1, select_13/1, select_03/1
  select_03/1 -> MMul_add_013/1
  select_13/1 -> MMul_add_013/2
  MMul_add_013/1 -> MMul_add_123/1
  select_23/1 -> MMul_add_123/2
  MMul_add_123/1 -> reshape_mmulResult3/1
  Gain4_const3/1 -> t14/1
  t15/1 -> vectorized_in04/1
  vectorized_in04/1 -> select_indices04/1
  select_indices04/1 -> Row2Col_in04/1
  select_indices14/1 -> Row2Col_in14/1
  delayMatch34/1 -> MMul_dot_product4/1(in0)
  Row2Col_in14/1 -> MMul_dot_product4/2(in1)
  MMul_dot_product_out_dtc4/1 -> reshape_dotProduct4/1
  reshape_dotProduct4/1 -> select_24/1, select_14/1, select_04/1
  select_04/1 -> MMul_add_014/1
  select_14/1 -> MMul_add_014/2
  MMul_add_014/1 -> MMul_add_124/1
  select_24/1 -> MMul_add_124/2
  MMul_add_124/1 -> reshape_mmulResult4/1
  Gain4_const4/1 -> t15/1
  t16/1 -> vectorized_in05/1
  vectorized_in05/1 -> select_indices05/1
  select_indices05/1 -> Row2Col_in05/1
  select_indices15/1 -> Row2Col_in15/1
  delayMatch39/1 -> MMul_dot_product5/1(in0)
  Row2Col_in15/1 -> MMul_dot_product5/2(in1)
  MMul_dot_product_out_dtc5/1 -> reshape_dotProduct5/1
  reshape_dotProduct5/1 -> select_25/1, select_15/1, select_05/1
  select_05/1 -> MMul_add_015/1
  select_15/1 -> MMul_add_015/2
  MMul_add_015/1 -> MMul_add_125/1
  select_25/1 -> MMul_add_125/2
  MMul_add_125/1 -> reshape_mmulResult5/1
  Gain4_const5/1 -> t16/1
  t17/1 -> t18/1(in0)
  t18/1(out0) -> t25/1
  t18/2(out1) -> t27/1
  t18/3(out2) -> t29/1
  t18/4(out3) -> t31/1
  t18/5(out4) -> t33/1
  t18/6(out5) -> t35/1
  t18/7(out6) -> t37/1
  t18/8(out7) -> t39/1
  t18/9(out8) -> t41/1
  _adder_MultiplyAdd_out_dtc8/1 -> t19/1
  _adder_MultiplyAdd_out_dtc17/1 -> t19/2
  _adder_MultiplyAdd_out_dtc26/1 -> t19/3
  _adder_MultiplyAdd_out_dtc35/1 -> t19/4
  _adder_MultiplyAdd_out_dtc44/1 -> t19/5
  _adder_MultiplyAdd_out_dtc53/1 -> t19/6
  _adder_MultiplyAdd_out_dtc62/1 -> t19/7
  _adder_MultiplyAdd_out_dtc71/1 -> t19/8
  _adder_MultiplyAdd_out_dtc80/1 -> t19/9
  t19/1 -> t20/1
  t21/1 -> t22/1(in0)
  delayMatch13/1 -> crp_temp_MAC2/1(in0)
  delayMatch14/1 -> crp_temp_MAC1/1(in0)
  delayMatch15/1 -> crp_temp_MAC5/1(in0)
  delayMatch16/1 -> crp_temp_MAC6/1(in0)
  delayMatch17/1 -> crp_temp_MAC7/1(in0)
  delayMatch18/1 -> crp_temp_MAC8/1(in0)
  delayMatch19/1 -> crp_temp_MAC/1(in0)
  delayMatch20/1 -> crp_temp_MAC3/1(in0)
  delayMatch21/1 -> crp_temp_MAC4/1(in0)
  crp_temp_MAC2/1(out0) -> t23/1
  crp_temp_MAC1/1(out0) -> t23/2
  crp_temp_MAC5/1(out0) -> t23/3
  crp_temp_MAC6/1(out0) -> t23/4
  crp_temp_MAC7/1(out0) -> t23/5
  crp_temp_MAC8/1(out0) -> t23/6
  crp_temp_MAC/1(out0) -> t23/7
  crp_temp_MAC3/1(out0) -> t23/8
  crp_temp_MAC4/1(out0) -> t23/9
  t23/1 -> t24/1
  _bias/1 -> _adder_MultiplyAdd/3(in2)
  delayMatch40/1 -> _adder_MultiplyAdd/1(in0)
  t26/1 -> _adder_MultiplyAdd/2(in1)
  delayMatch41/1 -> _adder_MultiplyAdd1/1(in0)
  _adder_MultiplyAdd_out_dtc/1 -> _adder_MultiplyAdd1/3(in2)
  delayMatch42/1 -> _adder_MultiplyAdd2/1(in0)
  _adder_MultiplyAdd_out_dtc1/1 -> _adder_MultiplyAdd2/3(in2)
  delayMatch43/1 -> _adder_MultiplyAdd3/1(in0)
  _adder_MultiplyAdd_out_dtc2/1 -> _adder_MultiplyAdd3/3(in2)
  delayMatch44/1 -> _adder_MultiplyAdd4/1(in0)
  _adder_MultiplyAdd_out_dtc3/1 -> _adder_MultiplyAdd4/3(in2)
  delayMatch45/1 -> _adder_MultiplyAdd5/1(in0)
  _adder_MultiplyAdd_out_dtc4/1 -> _adder_MultiplyAdd5/3(in2)
  delayMatch46/1 -> _adder_MultiplyAdd6/1(in0)
  _adder_MultiplyAdd_out_dtc5/1 -> _adder_MultiplyAdd6/3(in2)
  delayMatch47/1 -> _adder_MultiplyAdd7/1(in0)
  _adder_MultiplyAdd_out_dtc6/1 -> _adder_MultiplyAdd7/3(in2)
  delayMatch112/1 -> _adder_MultiplyAdd8/1(in0)
  _adder_MultiplyAdd_out_dtc7/1 -> _adder_MultiplyAdd8/3(in2)
  _bias1/1 -> _adder_MultiplyAdd9/3(in2)
  delayMatch48/1 -> _adder_MultiplyAdd9/1(in0)
  t28/1 -> _adder_MultiplyAdd9/2(in1)
  delayMatch49/1 -> _adder_MultiplyAdd10/1(in0)
  _adder_MultiplyAdd_out_dtc9/1 -> _adder_MultiplyAdd10/3(in2)
  delayMatch50/1 -> _adder_MultiplyAdd11/1(in0)
  _adder_MultiplyAdd_out_dtc10/1 -> _adder_MultiplyAdd11/3(in2)
  delayMatch51/1 -> _adder_MultiplyAdd12/1(in0)
  _adder_MultiplyAdd_out_dtc11/1 -> _adder_MultiplyAdd12/3(in2)
  delayMatch52/1 -> _adder_MultiplyAdd13/1(in0)
  _adder_MultiplyAdd_out_dtc12/1 -> _adder_MultiplyAdd13/3(in2)
  delayMatch53/1 -> _adder_MultiplyAdd14/1(in0)
  _adder_MultiplyAdd_out_dtc13/1 -> _adder_MultiplyAdd14/3(in2)
  delayMatch54/1 -> _adder_MultiplyAdd15/1(in0)
  _adder_MultiplyAdd_out_dtc14/1 -> _adder_MultiplyAdd15/3(in2)
  delayMatch55/1 -> _adder_MultiplyAdd16/1(in0)
  _adder_MultiplyAdd_out_dtc15/1 -> _adder_MultiplyAdd16/3(in2)
  delayMatch113/1 -> _adder_MultiplyAdd17/1(in0)
  _adder_MultiplyAdd_out_dtc16/1 -> _adder_MultiplyAdd17/3(in2)
  _bias2/1 -> _adder_MultiplyAdd18/3(in2)
  delayMatch56/1 -> _adder_MultiplyAdd18/1(in0)
  t30/1 -> _adder_MultiplyAdd18/2(in1)
  delayMatch57/1 -> _adder_MultiplyAdd19/1(in0)
  _adder_MultiplyAdd_out_dtc18/1 -> _adder_MultiplyAdd19/3(in2)
  delayMatch58/1 -> _adder_MultiplyAdd20/1(in0)
  _adder_MultiplyAdd_out_dtc19/1 -> _adder_MultiplyAdd20/3(in2)
  delayMatch59/1 -> _adder_MultiplyAdd21/1(in0)
  _adder_MultiplyAdd_out_dtc20/1 -> _adder_MultiplyAdd21/3(in2)
  delayMatch60/1 -> _adder_MultiplyAdd22/1(in0)
  _adder_MultiplyAdd_out_dtc21/1 -> _adder_MultiplyAdd22/3(in2)
  delayMatch61/1 -> _adder_MultiplyAdd23/1(in0)
  _adder_MultiplyAdd_out_dtc22/1 -> _adder_MultiplyAdd23/3(in2)
  delayMatch62/1 -> _adder_MultiplyAdd24/1(in0)
  _adder_MultiplyAdd_out_dtc23/1 -> _adder_MultiplyAdd24/3(in2)
  delayMatch63/1 -> _adder_MultiplyAdd25/1(in0)
  _adder_MultiplyAdd_out_dtc24/1 -> _adder_MultiplyAdd25/3(in2)
  delayMatch114/1 -> _adder_MultiplyAdd26/1(in0)
  _adder_MultiplyAdd_out_dtc25/1 -> _adder_MultiplyAdd26/3(in2)
  _bias3/1 -> _adder_MultiplyAdd27/3(in2)
  delayMatch64/1 -> _adder_MultiplyAdd27/1(in0)
  t32/1 -> _adder_MultiplyAdd27/2(in1)
  delayMatch65/1 -> _adder_MultiplyAdd28/1(in0)
  _adder_MultiplyAdd_out_dtc27/1 -> _adder_MultiplyAdd28/3(in2)
  delayMatch66/1 -> _adder_MultiplyAdd29/1(in0)
  _adder_MultiplyAdd_out_dtc28/1 -> _adder_MultiplyAdd29/3(in2)
  delayMatch67/1 -> _adder_MultiplyAdd30/1(in0)
  _adder_MultiplyAdd_out_dtc29/1 -> _adder_MultiplyAdd30/3(in2)
  delayMatch68/1 -> _adder_MultiplyAdd31/1(in0)
  _adder_MultiplyAdd_out_dtc30/1 -> _adder_MultiplyAdd31/3(in2)
  delayMatch69/1 -> _adder_MultiplyAdd32/1(in0)
  _adder_MultiplyAdd_out_dtc31/1 -> _adder_MultiplyAdd32/3(in2)
  delayMatch70/1 -> _adder_MultiplyAdd33/1(in0)
  _adder_MultiplyAdd_out_dtc32/1 -> _adder_MultiplyAdd33/3(in2)
  delayMatch71/1 -> _adder_MultiplyAdd34/1(in0)
  _adder_MultiplyAdd_out_dtc33/1 -> _adder_MultiplyAdd34/3(in2)
  delayMatch115/1 -> _adder_MultiplyAdd35/1(in0)
  _adder_MultiplyAdd_out_dtc34/1 -> _adder_MultiplyAdd35/3(in2)
  _bias4/1 -> _adder_MultiplyAdd36/3(in2)
  delayMatch72/1 -> _adder_MultiplyAdd36/1(in0)
  t34/1 -> _adder_MultiplyAdd36/2(in1)
  delayMatch73/1 -> _adder_MultiplyAdd37/1(in0)
  _adder_MultiplyAdd_out_dtc36/1 -> _adder_MultiplyAdd37/3(in2)
  delayMatch74/1 -> _adder_MultiplyAdd38/1(in0)
  _adder_MultiplyAdd_out_dtc37/1 -> _adder_MultiplyAdd38/3(in2)
  delayMatch75/1 -> _adder_MultiplyAdd39/1(in0)
  _adder_MultiplyAdd_out_dtc38/1 -> _adder_MultiplyAdd39/3(in2)
  delayMatch76/1 -> _adder_MultiplyAdd40/1(in0)
  _adder_MultiplyAdd_out_dtc39/1 -> _adder_MultiplyAdd40/3(in2)
  delayMatch77/1 -> _adder_MultiplyAdd41/1(in0)
  _adder_MultiplyAdd_out_dtc40/1 -> _adder_MultiplyAdd41/3(in2)
  delayMatch78/1 -> _adder_MultiplyAdd42/1(in0)
  _adder_MultiplyAdd_out_dtc41/1 -> _adder_MultiplyAdd42/3(in2)
  delayMatch79/1 -> _adder_MultiplyAdd43/1(in0)
  _adder_MultiplyAdd_out_dtc42/1 -> _adder_MultiplyAdd43/3(in2)
  delayMatch116/1 -> _adder_MultiplyAdd44/1(in0)
  _adder_MultiplyAdd_out_dtc43/1 -> _adder_MultiplyAdd44/3(in2)
  _bias5/1 -> _adder_MultiplyAdd45/3(in2)
  delayMatch80/1 -> _adder_MultiplyAdd45/1(in0)
  t36/1 -> _adder_MultiplyAdd45/2(in1)
  delayMatch81/1 -> _adder_MultiplyAdd46/1(in0)
  _adder_MultiplyAdd_out_dtc45/1 -> _adder_MultiplyAdd46/3(in2)
  delayMatch82/1 -> _adder_MultiplyAdd47/1(in0)
  _adder_MultiplyAdd_out_dtc46/1 -> _adder_MultiplyAdd47/3(in2)
  delayMatch83/1 -> _adder_MultiplyAdd48/1(in0)
  _adder_MultiplyAdd_out_dtc47/1 -> _adder_MultiplyAdd48/3(in2)
  delayMatch84/1 -> _adder_MultiplyAdd49/1(in0)
  _adder_MultiplyAdd_out_dtc48/1 -> _adder_MultiplyAdd49/3(in2)
  delayMatch85/1 -> _adder_MultiplyAdd50/1(in0)
  _adder_MultiplyAdd_out_dtc49/1 -> _adder_MultiplyAdd50/3(in2)
  delayMatch86/1 -> _adder_MultiplyAdd51/1(in0)
  _adder_MultiplyAdd_out_dtc50/1 -> _adder_MultiplyAdd51/3(in2)
  delayMatch87/1 -> _adder_MultiplyAdd52/1(in0)
  _adder_MultiplyAdd_out_dtc51/1 -> _adder_MultiplyAdd52/3(in2)
  delayMatch117/1 -> _adder_MultiplyAdd53/1(in0)
  _adder_MultiplyAdd_out_dtc52/1 -> _adder_MultiplyAdd53/3(in2)
  _bias6/1 -> _adder_MultiplyAdd54/3(in2)
  delayMatch88/1 -> _adder_MultiplyAdd54/1(in0)
  t38/1 -> _adder_MultiplyAdd54/2(in1)
  delayMatch89/1 -> _adder_MultiplyAdd55/1(in0)
  _adder_MultiplyAdd_out_dtc54/1 -> _adder_MultiplyAdd55/3(in2)
  delayMatch90/1 -> _adder_MultiplyAdd56/1(in0)
  _adder_MultiplyAdd_out_dtc55/1 -> _adder_MultiplyAdd56/3(in2)
  delayMatch91/1 -> _adder_MultiplyAdd57/1(in0)
  _adder_MultiplyAdd_out_dtc56/1 -> _adder_MultiplyAdd57/3(in2)
  delayMatch92/1 -> _adder_MultiplyAdd58/1(in0)
  _adder_MultiplyAdd_out_dtc57/1 -> _adder_MultiplyAdd58/3(in2)
  delayMatch93/1 -> _adder_MultiplyAdd59/1(in0)
  _adder_MultiplyAdd_out_dtc58/1 -> _adder_MultiplyAdd59/3(in2)
  delayMatch94/1 -> _adder_MultiplyAdd60/1(in0)
  _adder_MultiplyAdd_out_dtc59/1 -> _adder_MultiplyAdd60/3(in2)
  delayMatch95/1 -> _adder_MultiplyAdd61/1(in0)
  _adder_MultiplyAdd_out_dtc60/1 -> _adder_MultiplyAdd61/3(in2)
  delayMatch118/1 -> _adder_MultiplyAdd62/1(in0)
  _adder_MultiplyAdd_out_dtc61/1 -> _adder_MultiplyAdd62/3(in2)
  _bias7/1 -> _adder_MultiplyAdd63/3(in2)
  delayMatch96/1 -> _adder_MultiplyAdd63/1(in0)
  t40/1 -> _adder_MultiplyAdd63/2(in1)
  delayMatch97/1 -> _adder_MultiplyAdd64/1(in0)
  _adder_MultiplyAdd_out_dtc63/1 -> _adder_MultiplyAdd64/3(in2)
  delayMatch98/1 -> _adder_MultiplyAdd65/1(in0)
  _adder_MultiplyAdd_out_dtc64/1 -> _adder_MultiplyAdd65/3(in2)
  delayMatch99/1 -> _adder_MultiplyAdd66/1(in0)
  _adder_MultiplyAdd_out_dtc65/1 -> _adder_MultiplyAdd66/3(in2)
  delayMatch100/1 -> _adder_MultiplyAdd67/1(in0)
  _adder_MultiplyAdd_out_dtc66/1 -> _adder_MultiplyAdd67/3(in2)
  delayMatch101/1 -> _adder_MultiplyAdd68/1(in0)
  _adder_MultiplyAdd_out_dtc67/1 -> _adder_MultiplyAdd68/3(in2)
  delayMatch102/1 -> _adder_MultiplyAdd69/1(in0)
  _adder_MultiplyAdd_out_dtc68/1 -> _adder_MultiplyAdd69/3(in2)
  delayMatch103/1 -> _adder_MultiplyAdd70/1(in0)
  _adder_MultiplyAdd_out_dtc69/1 -> _adder_MultiplyAdd70/3(in2)
  delayMatch119/1 -> _adder_MultiplyAdd71/1(in0)
  _adder_MultiplyAdd_out_dtc70/1 -> _adder_MultiplyAdd71/3(in2)
  _bias8/1 -> _adder_MultiplyAdd72/3(in2)
  delayMatch104/1 -> _adder_MultiplyAdd72/1(in0)
  t42/1 -> _adder_MultiplyAdd72/2(in1)
  delayMatch105/1 -> _adder_MultiplyAdd73/1(in0)
  _adder_MultiplyAdd_out_dtc72/1 -> _adder_MultiplyAdd73/3(in2)
  delayMatch106/1 -> _adder_MultiplyAdd74/1(in0)
  _adder_MultiplyAdd_out_dtc73/1 -> _adder_MultiplyAdd74/3(in2)
  delayMatch107/1 -> _adder_MultiplyAdd75/1(in0)
  _adder_MultiplyAdd_out_dtc74/1 -> _adder_MultiplyAdd75/3(in2)
  delayMatch108/1 -> _adder_MultiplyAdd76/1(in0)
  _adder_MultiplyAdd_out_dtc75/1 -> _adder_MultiplyAdd76/3(in2)
  delayMatch109/1 -> _adder_MultiplyAdd77/1(in0)
  _adder_MultiplyAdd_out_dtc76/1 -> _adder_MultiplyAdd77/3(in2)
  delayMatch110/1 -> _adder_MultiplyAdd78/1(in0)
  _adder_MultiplyAdd_out_dtc77/1 -> _adder_MultiplyAdd78/3(in2)
  delayMatch111/1 -> _adder_MultiplyAdd79/1(in0)
  _adder_MultiplyAdd_out_dtc78/1 -> _adder_MultiplyAdd79/3(in2)
  delayMatch120/1 -> _adder_MultiplyAdd80/1(in0)
  _adder_MultiplyAdd_out_dtc79/1 -> _adder_MultiplyAdd80/3(in2)
  Gain_const/1 -> Gain/1(in0)
  Gain2_const/1 -> Gain2/2(in1)
  Gain2_const1/1 -> Gain21/2(in1)
  Gain2_const2/1 -> Gain22/2(in1)
  Product_C2ReIm_1/1 -> Product/1(in0), Product1/1(in0)
  Product_C2ReIm_1/2 -> Product2/1(in0), Product3/1(in0)
  delayMatch23/1 -> Product/2(in1)
  delayMatch24/1 -> Product1/2(in1)
  Product/1(out0) -> Product_AC_minus_BD/1
  Product1/1(out0) -> Product_AD_plus_BC/1
  Product2/1(out0) -> Product_AC_minus_BD/2
  Product3/1(out0) -> Product_AD_plus_BC/2
  Product_AC_minus_BD/1 -> Product_ReIm2Complex/1
  Product_AD_plus_BC/1 -> Product_ReIm2Complex/2
  Product_C2ReIm_11/1 -> Product4/1(in0), Product5/1(in0)
  Product_C2ReIm_11/2 -> Product6/1(in0), Product7/1(in0)
  delayMatch29/1 -> Product4/2(in1)
  delayMatch30/1 -> Product5/2(in1)
  Product4/1(out0) -> Product_AC_minus_BD1/1
  Product5/1(out0) -> Product_AD_plus_BC1/1
  Product6/1(out0) -> Product_AC_minus_BD1/2
  Product7/1(out0) -> Product_AD_plus_BC1/2
  Product_AC_minus_BD1/1 -> Product_ReIm2Complex1/1
  Product_AD_plus_BC1/1 -> Product_ReIm2Complex1/2
  Product_C2ReIm_12/1 -> Product8/1(in0), Product9/1(in0)
  Product_C2ReIm_12/2 -> Product10/1(in0), Product11/1(in0)
  delayMatch35/1 -> Product8/2(in1)
  delayMatch36/1 -> Product9/2(in1)
  Product8/1(out0) -> Product_AC_minus_BD2/1
  Product9/1(out0) -> Product_AD_plus_BC2/1
  Product10/1(out0) -> Product_AC_minus_BD2/2
  Product11/1(out0) -> Product_AD_plus_BC2/2
  Product_AC_minus_BD2/1 -> Product_ReIm2Complex2/1
  Product_AD_plus_BC2/1 -> Product_ReIm2Complex2/2
  MMul_dot_product/1(out0) -> MMul_dot_product_out_dtc/1
  MMul_dot_product1/1(out0) -> MMul_dot_product_out_dtc1/1
  MMul_dot_product2/1(out0) -> MMul_dot_product_out_dtc2/1
  MMul_dot_product3/1(out0) -> MMul_dot_product_out_dtc3/1
  MMul_dot_product4/1(out0) -> MMul_dot_product_out_dtc4/1
  MMul_dot_product5/1(out0) -> MMul_dot_product_out_dtc5/1
  _adder_MultiplyAdd/1(out0) -> _adder_MultiplyAdd_out_dtc/1
  _adder_MultiplyAdd1/1(out0) -> _adder_MultiplyAdd_out_dtc1/1
  _adder_MultiplyAdd2/1(out0) -> _adder_MultiplyAdd_out_dtc2/1
  _adder_MultiplyAdd3/1(out0) -> _adder_MultiplyAdd_out_dtc3/1
  _adder_MultiplyAdd4/1(out0) -> _adder_MultiplyAdd_out_dtc4/1
  _adder_MultiplyAdd5/1(out0) -> _adder_MultiplyAdd_out_dtc5/1
  _adder_MultiplyAdd6/1(out0) -> _adder_MultiplyAdd_out_dtc6/1
  _adder_MultiplyAdd7/1(out0) -> _adder_MultiplyAdd_out_dtc7/1
  _adder_MultiplyAdd8/1(out0) -> _adder_MultiplyAdd_out_dtc8/1
  _adder_MultiplyAdd9/1(out0) -> _adder_MultiplyAdd_out_dtc9/1
  _adder_MultiplyAdd10/1(out0) -> _adder_MultiplyAdd_out_dtc10/1
  _adder_MultiplyAdd11/1(out0) -> _adder_MultiplyAdd_out_dtc11/1
  _adder_MultiplyAdd12/1(out0) -> _adder_MultiplyAdd_out_dtc12/1
  _adder_MultiplyAdd13/1(out0) -> _adder_MultiplyAdd_out_dtc13/1
  _adder_MultiplyAdd14/1(out0) -> _adder_MultiplyAdd_out_dtc14/1
  _adder_MultiplyAdd15/1(out0) -> _adder_MultiplyAdd_out_dtc15/1
  _adder_MultiplyAdd16/1(out0) -> _adder_MultiplyAdd_out_dtc16/1
  _adder_MultiplyAdd17/1(out0) -> _adder_MultiplyAdd_out_dtc17/1
  _adder_MultiplyAdd18/1(out0) -> _adder_MultiplyAdd_out_dtc18/1
  _adder_MultiplyAdd19/1(out0) -> _adder_MultiplyAdd_out_dtc19/1
  _adder_MultiplyAdd20/1(out0) -> _adder_MultiplyAdd_out_dtc20/1
  _adder_MultiplyAdd21/1(out0) -> _adder_MultiplyAdd_out_dtc21/1
  _adder_MultiplyAdd22/1(out0) -> _adder_MultiplyAdd_out_dtc22/1
  _adder_MultiplyAdd23/1(out0) -> _adder_MultiplyAdd_out_dtc23/1
  _adder_MultiplyAdd24/1(out0) -> _adder_MultiplyAdd_out_dtc24/1
  _adder_MultiplyAdd25/1(out0) -> _adder_MultiplyAdd_out_dtc25/1
  _adder_MultiplyAdd26/1(out0) -> _adder_MultiplyAdd_out_dtc26/1
  _adder_MultiplyAdd27/1(out0) -> _adder_MultiplyAdd_out_dtc27/1
  _adder_MultiplyAdd28/1(out0) -> _adder_MultiplyAdd_out_dtc28/1
  _adder_MultiplyAdd29/1(out0) -> _adder_MultiplyAdd_out_dtc29/1
  _adder_MultiplyAdd30/1(out0) -> _adder_MultiplyAdd_out_dtc30/1
  _adder_MultiplyAdd31/1(out0) -> _adder_MultiplyAdd_out_dtc31/1
  _adder_MultiplyAdd32/1(out0) -> _adder_MultiplyAdd_out_dtc32/1
  _adder_MultiplyAdd33/1(out0) -> _adder_MultiplyAdd_out_dtc33/1
  _adder_MultiplyAdd34/1(out0) -> _adder_MultiplyAdd_out_dtc34/1
  _adder_MultiplyAdd35/1(out0) -> _adder_MultiplyAdd_out_dtc35/1
  _adder_MultiplyAdd36/1(out0) -> _adder_MultiplyAdd_out_dtc36/1
  _adder_MultiplyAdd37/1(out0) -> _adder_MultiplyAdd_out_dtc37/1
  _adder_MultiplyAdd38/1(out0) -> _adder_MultiplyAdd_out_dtc38/1
  _adder_MultiplyAdd39/1(out0) -> _adder_MultiplyAdd_out_dtc39/1
  _adder_MultiplyAdd40/1(out0) -> _adder_MultiplyAdd_out_dtc40/1
  _adder_MultiplyAdd41/1(out0) -> _adder_MultiplyAdd_out_dtc41/1
  _adder_MultiplyAdd42/1(out0) -> _adder_MultiplyAdd_out_dtc42/1
  _adder_MultiplyAdd43/1(out0) -> _adder_MultiplyAdd_out_dtc43/1
  _adder_MultiplyAdd44/1(out0) -> _adder_MultiplyAdd_out_dtc44/1
  _adder_MultiplyAdd45/1(out0) -> _adder_MultiplyAdd_out_dtc45/1
  _adder_MultiplyAdd46/1(out0) -> _adder_MultiplyAdd_out_dtc46/1
  _adder_MultiplyAdd47/1(out0) -> _adder_MultiplyAdd_out_dtc47/1
  _adder_MultiplyAdd48/1(out0) -> _adder_MultiplyAdd_out_dtc48/1
  _adder_MultiplyAdd49/1(out0) -> _adder_MultiplyAdd_out_dtc49/1
  _adder_MultiplyAdd50/1(out0) -> _adder_MultiplyAdd_out_dtc50/1
  _adder_MultiplyAdd51/1(out0) -> _adder_MultiplyAdd_out_dtc51/1
  _adder_MultiplyAdd52/1(out0) -> _adder_MultiplyAdd_out_dtc52/1
  _adder_MultiplyAdd53/1(out0) -> _adder_MultiplyAdd_out_dtc53/1
  _adder_MultiplyAdd54/1(out0) -> _adder_MultiplyAdd_out_dtc54/1
  _adder_MultiplyAdd55/1(out0) -> _adder_MultiplyAdd_out_dtc55/1
  _adder_MultiplyAdd56/1(out0) -> _adder_MultiplyAdd_out_dtc56/1
  _adder_MultiplyAdd57/1(out0) -> _adder_MultiplyAdd_out_dtc57/1
  _adder_MultiplyAdd58/1(out0) -> _adder_MultiplyAdd_out_dtc58/1
  _adder_MultiplyAdd59/1(out0) -> _adder_MultiplyAdd_out_dtc59/1
  _adder_MultiplyAdd60/1(out0) -> _adder_MultiplyAdd_out_dtc60/1
  _adder_MultiplyAdd61/1(out0) -> _adder_MultiplyAdd_out_dtc61/1
  _adder_MultiplyAdd62/1(out0) -> _adder_MultiplyAdd_out_dtc62/1
  _adder_MultiplyAdd63/1(out0) -> _adder_MultiplyAdd_out_dtc63/1
  _adder_MultiplyAdd64/1(out0) -> _adder_MultiplyAdd_out_dtc64/1
  _adder_MultiplyAdd65/1(out0) -> _adder_MultiplyAdd_out_dtc65/1
  _adder_MultiplyAdd66/1(out0) -> _adder_MultiplyAdd_out_dtc66/1
  _adder_MultiplyAdd67/1(out0) -> _adder_MultiplyAdd_out_dtc67/1
  _adder_MultiplyAdd68/1(out0) -> _adder_MultiplyAdd_out_dtc68/1
  _adder_MultiplyAdd69/1(out0) -> _adder_MultiplyAdd_out_dtc69/1
  _adder_MultiplyAdd70/1(out0) -> _adder_MultiplyAdd_out_dtc70/1
  _adder_MultiplyAdd71/1(out0) -> _adder_MultiplyAdd_out_dtc71/1
  _adder_MultiplyAdd72/1(out0) -> _adder_MultiplyAdd_out_dtc72/1
  _adder_MultiplyAdd73/1(out0) -> _adder_MultiplyAdd_out_dtc73/1
  _adder_MultiplyAdd74/1(out0) -> _adder_MultiplyAdd_out_dtc74/1
  _adder_MultiplyAdd75/1(out0) -> _adder_MultiplyAdd_out_dtc75/1
  _adder_MultiplyAdd76/1(out0) -> _adder_MultiplyAdd_out_dtc76/1
  _adder_MultiplyAdd77/1(out0) -> _adder_MultiplyAdd_out_dtc77/1
  _adder_MultiplyAdd78/1(out0) -> _adder_MultiplyAdd_out_dtc78/1
  _adder_MultiplyAdd79/1(out0) -> _adder_MultiplyAdd_out_dtc79/1
  _adder_MultiplyAdd80/1(out0) -> _adder_MultiplyAdd_out_dtc80/1
  Gain2/1(out0) -> Gain2_out_dtc/1
  Gain21/1(out0) -> Gain2_out_dtc1/1
  Gain22/1(out0) -> Gain2_out_dtc2/1
  delayMatch3/1 -> Divide2/2(in1)
  x_in_dq_0_wire/1 -> delayMatch3/1, delayMatch2/1
  delayMatch5/1 -> Divide3/2(in1)
  x_in_dq_1_wire/1 -> delayMatch5/1, delayMatch4/1
  t22/1(out0) -> delayMatch13/1
  t22/2(out1) -> delayMatch14/1
  t22/3(out2) -> delayMatch15/1
  t22/4(out3) -> delayMatch16/1
  t22/5(out4) -> delayMatch17/1
  t22/6(out5) -> delayMatch18/1
  t22/7(out6) -> delayMatch19/1
  t22/8(out7) -> delayMatch20/1
  t22/9(out8) -> delayMatch21/1
  Row2Col_in0/1 -> delayMatch22/1
  delayMatch26/1 -> Product3/2(in1)
  delayMatch25/1 -> Product2/2(in1)
  Product_C2ReIm_2/2 -> delayMatch25/1, delayMatch24/1
  Product_C2ReIm_2/1 -> delayMatch26/1, delayMatch23/1
  Row2Col_in01/1 -> delayMatch27/1
  Row2Col_in02/1 -> delayMatch28/1
  delayMatch32/1 -> Product7/2(in1)
  delayMatch31/1 -> Product6/2(in1)
  Product_C2ReIm_21/2 -> delayMatch31/1, delayMatch30/1
  Product_C2ReIm_21/1 -> delayMatch32/1, delayMatch29/1
  Row2Col_in03/1 -> delayMatch33/1
  Row2Col_in04/1 -> delayMatch34/1
  delayMatch38/1 -> Product11/2(in1)
  delayMatch37/1 -> Product10/2(in1)
  Product_C2ReIm_22/2 -> delayMatch37/1, delayMatch36/1
  Product_C2ReIm_22/1 -> delayMatch38/1, delayMatch35/1
  Row2Col_in05/1 -> delayMatch39/1
  t25/1 -> delayMatch40/1
  t25/2 -> delayMatch41/1
  t26/2 -> _adder_MultiplyAdd1/2(in1)
  t25/3 -> delayMatch42/1
  t26/3 -> _adder_MultiplyAdd2/2(in1)
  t25/4 -> delayMatch43/1
  t26/4 -> _adder_MultiplyAdd3/2(in1)
  t25/5 -> delayMatch44/1
  t26/5 -> _adder_MultiplyAdd4/2(in1)
  t25/6 -> delayMatch45/1
  t26/6 -> _adder_MultiplyAdd5/2(in1)
  t25/7 -> delayMatch46/1
  t26/7 -> _adder_MultiplyAdd6/2(in1)
  t25/8 -> delayMatch47/1
  t26/8 -> _adder_MultiplyAdd7/2(in1)
  t27/1 -> delayMatch48/1
  t27/2 -> delayMatch49/1
  t28/2 -> _adder_MultiplyAdd10/2(in1)
  t27/3 -> delayMatch50/1
  t28/3 -> _adder_MultiplyAdd11/2(in1)
  t27/4 -> delayMatch51/1
  t28/4 -> _adder_MultiplyAdd12/2(in1)
  t27/5 -> delayMatch52/1
  t28/5 -> _adder_MultiplyAdd13/2(in1)
  t27/6 -> delayMatch53/1
  t28/6 -> _adder_MultiplyAdd14/2(in1)
  t27/7 -> delayMatch54/1
  t28/7 -> _adder_MultiplyAdd15/2(in1)
  t27/8 -> delayMatch55/1
  t28/8 -> _adder_MultiplyAdd16/2(in1)
  t29/1 -> delayMatch56/1
  t29/2 -> delayMatch57/1
  t30/2 -> _adder_MultiplyAdd19/2(in1)
  t29/3 -> delayMatch58/1
  t30/3 -> _adder_MultiplyAdd20/2(in1)
  t29/4 -> delayMatch59/1
  t30/4 -> _adder_MultiplyAdd21/2(in1)
  t29/5 -> delayMatch60/1
  t30/5 -> _adder_MultiplyAdd22/2(in1)
  t29/6 -> delayMatch61/1
  t30/6 -> _adder_MultiplyAdd23/2(in1)
  t29/7 -> delayMatch62/1
  t30/7 -> _adder_MultiplyAdd24/2(in1)
  t29/8 -> delayMatch63/1
  t30/8 -> _adder_MultiplyAdd25/2(in1)
  t31/1 -> delayMatch64/1
  t31/2 -> delayMatch65/1
  t32/2 -> _adder_MultiplyAdd28/2(in1)
  t31/3 -> delayMatch66/1
  t32/3 -> _adder_MultiplyAdd29/2(in1)
  t31/4 -> delayMatch67/1
  t32/4 -> _adder_MultiplyAdd30/2(in1)
  t31/5 -> delayMatch68/1
  t32/5 -> _adder_MultiplyAdd31/2(in1)
  t31/6 -> delayMatch69/1
  t32/6 -> _adder_MultiplyAdd32/2(in1)
  t31/7 -> delayMatch70/1
  t32/7 -> _adder_MultiplyAdd33/2(in1)
  t31/8 -> delayMatch71/1
  t32/8 -> _adder_MultiplyAdd34/2(in1)
  t33/1 -> delayMatch72/1
  t33/2 -> delayMatch73/1
  t34/2 -> _adder_MultiplyAdd37/2(in1)
  t33/3 -> delayMatch74/1
  t34/3 -> _adder_MultiplyAdd38/2(in1)
  t33/4 -> delayMatch75/1
  t34/4 -> _adder_MultiplyAdd39/2(in1)
  t33/5 -> delayMatch76/1
  t34/5 -> _adder_MultiplyAdd40/2(in1)
  t33/6 -> delayMatch77/1
  t34/6 -> _adder_MultiplyAdd41/2(in1)
  t33/7 -> delayMatch78/1
  t34/7 -> _adder_MultiplyAdd42/2(in1)
  t33/8 -> delayMatch79/1
  t34/8 -> _adder_MultiplyAdd43/2(in1)
  t35/1 -> delayMatch80/1
  t35/2 -> delayMatch81/1
  t36/2 -> _adder_MultiplyAdd46/2(in1)
  t35/3 -> delayMatch82/1
  t36/3 -> _adder_MultiplyAdd47/2(in1)
  t35/4 -> delayMatch83/1
  t36/4 -> _adder_MultiplyAdd48/2(in1)
  t35/5 -> delayMatch84/1
  t36/5 -> _adder_MultiplyAdd49/2(in1)
  t35/6 -> delayMatch85/1
  t36/6 -> _adder_MultiplyAdd50/2(in1)
  t35/7 -> delayMatch86/1
  t36/7 -> _adder_MultiplyAdd51/2(in1)
  t35/8 -> delayMatch87/1
  t36/8 -> _adder_MultiplyAdd52/2(in1)
  t37/1 -> delayMatch88/1
  t37/2 -> delayMatch89/1
  t38/2 -> _adder_MultiplyAdd55/2(in1)
  t37/3 -> delayMatch90/1
  t38/3 -> _adder_MultiplyAdd56/2(in1)
  t37/4 -> delayMatch91/1
  t38/4 -> _adder_MultiplyAdd57/2(in1)
  t37/5 -> delayMatch92/1
  t38/5 -> _adder_MultiplyAdd58/2(in1)
  t37/6 -> delayMatch93/1
  t38/6 -> _adder_MultiplyAdd59/2(in1)
  t37/7 -> delayMatch94/1
  t38/7 -> _adder_MultiplyAdd60/2(in1)
  t37/8 -> delayMatch95/1
  t38/8 -> _adder_MultiplyAdd61/2(in1)
  t39/1 -> delayMatch96/1
  t39/2 -> delayMatch97/1
  t40/2 -> _adder_MultiplyAdd64/2(in1)
  t39/3 -> delayMatch98/1
  t40/3 -> _adder_MultiplyAdd65/2(in1)
  t39/4 -> delayMatch99/1
  t40/4 -> _adder_MultiplyAdd66/2(in1)
  t39/5 -> delayMatch100/1
  t40/5 -> _adder_MultiplyAdd67/2(in1)
  t39/6 -> delayMatch101/1
  t40/6 -> _adder_MultiplyAdd68/2(in1)
  t39/7 -> delayMatch102/1
  t40/7 -> _adder_MultiplyAdd69/2(in1)
  t39/8 -> delayMatch103/1
  t40/8 -> _adder_MultiplyAdd70/2(in1)
  t41/1 -> delayMatch104/1
  t41/2 -> delayMatch105/1
  t42/2 -> _adder_MultiplyAdd73/2(in1)
  t41/3 -> delayMatch106/1
  t42/3 -> _adder_MultiplyAdd74/2(in1)
  t41/4 -> delayMatch107/1
  t42/4 -> _adder_MultiplyAdd75/2(in1)
  t41/5 -> delayMatch108/1
  t42/5 -> _adder_MultiplyAdd76/2(in1)
  t41/6 -> delayMatch109/1
  t42/6 -> _adder_MultiplyAdd77/2(in1)
  t41/7 -> delayMatch110/1
  t42/7 -> _adder_MultiplyAdd78/2(in1)
  t41/8 -> delayMatch111/1
  t42/8 -> _adder_MultiplyAdd79/2(in1)
  t25/9 -> delayMatch112/1
  t26/9 -> _adder_MultiplyAdd8/2(in1)
  t27/9 -> delayMatch113/1
  t28/9 -> _adder_MultiplyAdd17/2(in1)
  t29/9 -> delayMatch114/1
  t30/9 -> _adder_MultiplyAdd26/2(in1)
  t31/9 -> delayMatch115/1
  t32/9 -> _adder_MultiplyAdd35/2(in1)
  t33/9 -> delayMatch116/1
  t34/9 -> _adder_MultiplyAdd44/2(in1)
  t35/9 -> delayMatch117/1
  t36/9 -> _adder_MultiplyAdd53/2(in1)
  t37/9 -> delayMatch118/1
  t38/9 -> _adder_MultiplyAdd62/2(in1)
  t39/9 -> delayMatch119/1
  t40/9 -> _adder_MultiplyAdd71/2(in1)
  t41/9 -> delayMatch120/1
  t42/9 -> _adder_MultiplyAdd80/2(in1)
  From2/1 -> Divide/1(in0)
  From22/1 -> Divide31/1(in0)
  From3/1 -> Divide1/1(in0)
  From12/1 -> Divide21/1(in0)
  Demux1_mux_1/1 -> Demux1_out1/1
  Demux1_mux_2/1 -> Demux1_out2/1
  Demux1_mux_3/1 -> Demux1_out3/1
  Switch/1 -> Switch_out11/1, Switch_out1/1
  enb_counter_ge_5_and_enb_counter_le_13/1 -> crp_temp_MAC2/Enable, crp_temp_MAC1/Enable, crp_temp_MAC5/Enable, crp_temp_MAC6/Enable, crp_temp_MAC7/Enable, crp_temp_MAC8/Enable, crp_temp_MAC/Enable, crp_temp_MAC3/Enable, crp_temp_MAC4/Enable
  enb_counter_ge_35_and_enb_counter_le_37/1 -> Divide/Enable, Divide1/Enable, Divide31/Enable, Divide21/Enable
  enb_counter_ge_3_and_enb_counter_le_5/1 -> Divide4/Enable, Divide11/Enable, Divide2/Enable, Divide3/Enable
  enb_counter_ge_2_and_enb_counter_le_4/1 -> MMul_dot_product4/Enable, MMul_dot_product2/Enable, MMul_dot_product/Enable
  enb_counter_ge_6_and_enb_counter_le_8/1 -> MMul_dot_product1/Enable, MMul_dot_product3/Enable, MMul_dot_product5/Enable
  enb_counter_ge_8_and_enb_counter_le_11/1 -> _adder_MultiplyAdd/Enable, _adder_MultiplyAdd9/Enable, _adder_MultiplyAdd18/Enable, _adder_MultiplyAdd27/Enable, _adder_MultiplyAdd36/Enable, _adder_MultiplyAdd45/Enable, _adder_MultiplyAdd54/Enable, _adder_MultiplyAdd63/Enable, _adder_MultiplyAdd72/Enable
  enb_counter_ge_11_and_enb_counter_le_14/1 -> _adder_MultiplyAdd1/Enable, _adder_MultiplyAdd10/Enable, _adder_MultiplyAdd19/Enable, _adder_MultiplyAdd28/Enable, _adder_MultiplyAdd37/Enable, _adder_MultiplyAdd46/Enable, _adder_MultiplyAdd55/Enable, _adder_MultiplyAdd64/Enable, _adder_MultiplyAdd73/Enable
  enb_counter_ge_14_and_enb_counter_le_17/1 -> _adder_MultiplyAdd2/Enable, _adder_MultiplyAdd11/Enable, _adder_MultiplyAdd20/Enable, _adder_MultiplyAdd29/Enable, _adder_MultiplyAdd38/Enable, _adder_MultiplyAdd47/Enable, _adder_MultiplyAdd56/Enable, _adder_MultiplyAdd65/Enable, _adder_MultiplyAdd74/Enable
  enb_counter_ge_17_and_enb_counter_le_20/1 -> _adder_MultiplyAdd3/Enable, _adder_MultiplyAdd12/Enable, _adder_MultiplyAdd21/Enable, _adder_MultiplyAdd30/Enable, _adder_MultiplyAdd39/Enable, _adder_MultiplyAdd48/Enable, _adder_MultiplyAdd57/Enable, _adder_MultiplyAdd66/Enable, _adder_MultiplyAdd75/Enable
  enb_counter_ge_20_and_enb_counter_le_23/1 -> _adder_MultiplyAdd4/Enable, _adder_MultiplyAdd13/Enable, _adder_MultiplyAdd22/Enable, _adder_MultiplyAdd31/Enable, _adder_MultiplyAdd40/Enable, _adder_MultiplyAdd49/Enable, _adder_MultiplyAdd58/Enable, _adder_MultiplyAdd67/Enable, _adder_MultiplyAdd76/Enable
  enb_counter_ge_23_and_enb_counter_le_26/1 -> _adder_MultiplyAdd5/Enable, _adder_MultiplyAdd14/Enable, _adder_MultiplyAdd23/Enable, _adder_MultiplyAdd32/Enable, _adder_MultiplyAdd41/Enable, _adder_MultiplyAdd50/Enable, _adder_MultiplyAdd59/Enable, _adder_MultiplyAdd68/Enable, _adder_MultiplyAdd77/Enable
  enb_counter_ge_26_and_enb_counter_le_29/1 -> _adder_MultiplyAdd6/Enable, _adder_MultiplyAdd15/Enable, _adder_MultiplyAdd24/Enable, _adder_MultiplyAdd33/Enable, _adder_MultiplyAdd42/Enable, _adder_MultiplyAdd51/Enable, _adder_MultiplyAdd60/Enable, _adder_MultiplyAdd69/Enable, _adder_MultiplyAdd78/Enable
  enb_counter_ge_29_and_enb_counter_le_32/1 -> _adder_MultiplyAdd7/Enable, _adder_MultiplyAdd16/Enable, _adder_MultiplyAdd25/Enable, _adder_MultiplyAdd34/Enable, _adder_MultiplyAdd43/Enable, _adder_MultiplyAdd52/Enable, _adder_MultiplyAdd61/Enable, _adder_MultiplyAdd70/Enable, _adder_MultiplyAdd79/Enable
  enb_counter_ge_32_and_enb_counter_le_35/1 -> _adder_MultiplyAdd8/Enable, _adder_MultiplyAdd17/Enable, _adder_MultiplyAdd26/Enable, _adder_MultiplyAdd35/Enable, _adder_MultiplyAdd44/Enable, _adder_MultiplyAdd53/Enable, _adder_MultiplyAdd62/Enable, _adder_MultiplyAdd71/Enable, _adder_MultiplyAdd80/Enable
  enb_counter_le_2/1 -> Gain22/Enable, Gain21/Enable, Gain2/Enable, Gain/Enable
  enb_counter_ge_4_and_enb_counter_le_6/1 -> Product/Enable, Product2/Enable, Product1/Enable, Product3/Enable, Product4/Enable, Product6/Enable, Product5/Enable, Product7/Enable, Product8/Enable, Product10/Enable, Product9/Enable, Product11/Enable
  enb_counter_ge_2/1 -> enb_counter_ge_2_and_enb_counter_le_4/1
  enb_counter_le_4/1 -> enb_counter_ge_2_and_enb_counter_le_4/2
  enb_counter_ge_3/1 -> enb_counter_ge_3_and_enb_counter_le_5/1
  enb_counter_le_5/1 -> enb_counter_ge_3_and_enb_counter_le_5/2
  enb_counter_ge_4/1 -> enb_counter_ge_4_and_enb_counter_le_6/1
  enb_counter_le_6/1 -> enb_counter_ge_4_and_enb_counter_le_6/2
  enb_counter_ge_5/1 -> enb_counter_ge_5_and_enb_counter_le_13/1
  enb_counter_le_13/1 -> enb_counter_ge_5_and_enb_counter_le_13/2
  enb_counter_ge_6/1 -> enb_counter_ge_6_and_enb_counter_le_8/1
  enb_counter_le_8/1 -> enb_counter_ge_6_and_enb_counter_le_8/2
  enb_counter_ge_8/1 -> enb_counter_ge_8_and_enb_counter_le_11/1
  enb_counter_le_11/1 -> enb_counter_ge_8_and_enb_counter_le_11/2
  enb_counter_ge_11/1 -> enb_counter_ge_11_and_enb_counter_le_14/1
  enb_counter_le_14/1 -> enb_counter_ge_11_and_enb_counter_le_14/2
  enb_counter_ge_14/1 -> enb_counter_ge_14_and_enb_counter_le_17/1
  enb_counter_le_17/1 -> enb_counter_ge_14_and_enb_counter_le_17/2
  enb_counter_ge_17/1 -> enb_counter_ge_17_and_enb_counter_le_20/1
  enb_counter_le_20/1 -> enb_counter_ge_17_and_enb_counter_le_20/2
  enb_counter_ge_20/1 -> enb_counter_ge_20_and_enb_counter_le_23/1
  enb_counter_le_23/1 -> enb_counter_ge_20_and_enb_counter_le_23/2
  enb_counter_ge_23/1 -> enb_counter_ge_23_and_enb_counter_le_26/1
  enb_counter_le_26/1 -> enb_counter_ge_23_and_enb_counter_le_26/2
  enb_counter_ge_26/1 -> enb_counter_ge_26_and_enb_counter_le_29/1
  enb_counter_le_29/1 -> enb_counter_ge_26_and_enb_counter_le_29/2
  enb_counter_ge_29/1 -> enb_counter_ge_29_and_enb_counter_le_32/1
  enb_counter_le_32/1 -> enb_counter_ge_29_and_enb_counter_le_32/2
  enb_counter_ge_32/1 -> enb_counter_ge_32_and_enb_counter_le_35/1
  enb_counter_le_35/1 -> enb_counter_ge_32_and_enb_counter_le_35/2
  enb_counter_ge_35/1 -> enb_counter_ge_35_and_enb_counter_le_37/1
  enb_counter_le_37/1 -> enb_counter_ge_35_and_enb_counter_le_37/2
  ctr_99/1 -> enb_counter_le_37/1, enb_counter_ge_35/1, enb_counter_le_35/1, enb_counter_ge_32/1, enb_counter_le_32/1, enb_counter_ge_29/1, enb_counter_le_29/1, enb_counter_ge_26/1, enb_counter_le_26/1, enb_counter_ge_23/1, enb_counter_le_23/1, enb_counter_ge_20/1, enb_counter_le_20/1, enb_counter_ge_17/1, enb_counter_le_17/1, enb_counter_ge_14/1, enb_counter_le_14/1, enb_counter_ge_11/1, enb_counter_le_11/1, enb_counter_ge_8/1, enb_counter_le_8/1, enb_counter_ge_6/1, enb_counter_le_13/1, enb_counter_ge_5/1, enb_counter_le_6/1, enb_counter_ge_4/1, enb_counter_le_5/1, enb_counter_ge_3/1, enb_counter_le_4/1, enb_counter_ge_2/1, enb_counter_le_2/1
